simulink model "Adaptive_Control_KpKd"  (R2021b)
settings: Solver=VariableStepAuto  StartTime=0.0  StopTime=10  RelTol=1e-3
undefined symbols (not defined in the file or in its folder): coef_init, Kd, Kp, Kpi, Lambda, q_dq_init
(part 4 of 4)

== matlab function Adaptive_Control_KpKd/MATLAB Function1 ==
  data: q input; dq input; ddq input; Yb output; g input
function Yb = Yb_fun(q,dq,ddq,g)
%YB_FUN
%    YB = YB_FUN(Q1,Q2,Q3,Q4,Q5,Q6,DQ1,DQ2,DQ3,DQ4,DQ5,DQ6,DDQ1,DDQ2,DDQ3,DDQ4,DDQ5,DDQ6,G)

%    This function was generated by the Symbolic Math Toolbox version 8.7.
%    16-Mar-2022 17:09:26

q1 = q(1);
q2 = q(2);
q3 = q(3);
q4 = q(4);
q5 = q(5);
q6 = q(6);

dq1 = dq(1);
dq2 = dq(2);
dq3 = dq(3);
dq4 = dq(4);
dq5 = dq(5);
dq6 = dq(6);

ddq1 = ddq(1);
ddq2 = ddq(2);
ddq3 = ddq(3);
ddq4 = ddq(4);
ddq5 = ddq(5);
ddq6 = ddq(6);

t2 = cos(q1);
t3 = cos(q2);
t4 = cos(q4);
t5 = cos(q5);
t6 = cos(q6);
t7 = sin(q1);
t8 = sin(q2);
t9 = sin(q4);
t10 = sin(q5);
t11 = sin(q6);
t12 = dq1.^2;
t13 = dq2.^2;
t14 = dq4.^2;
t15 = dq5.^2;
t16 = dq6.^2;
t17 = q2.*2.0;
t18 = q4.*2.0;
t19 = q5.*2.0;
t20 = q6.*2.0;
t90 = q3.*5.0e+3;
t21 = cos(t17);
t22 = t3.^2;
t23 = t4.^2;
t24 = t5.^2;
t25 = t6.^2;
t26 = sin(t17);
t27 = sin(t18);
t28 = sin(t19);
t29 = sin(t20);
t30 = t8.^2;
t31 = t9.^2;
t32 = ddq1.*t3;
t33 = ddq2.*t3;
t34 = ddq2.*t4;
t35 = ddq4.*t5;
t36 = ddq5.*t4;
t37 = ddq5.*t5;
t38 = g.*t2;
t39 = ddq1.*t8;
t40 = ddq2.*t9;
t41 = ddq4.*t8;
t42 = ddq4.*t9;
t43 = ddq4.*t10;
t44 = ddq5.*t10;
t45 = dq2.*dq4.*t9;
t46 = dq2.*dq5.*t9;
t47 = dq4.*dq5.*t9;
t48 = dq1.*dq2.*t3;
t49 = dq1.*dq4.*t3;
t50 = dq2.*dq4.*t3;
t51 = dq4.*dq5.*t5;
t52 = dq4.*dq6.*t5;
t53 = dq5.*dq6.*t5;
t54 = t8.*t13;
t55 = t10.*t13;
t56 = t10.*t15;
t57 = dq2.*dq4.*t10.*2.0;
t58 = -t12;
t60 = ddq4.*t3.*t4;
t63 = ddq6.*t5.*t6;
t71 = ddq5.*t3.*t9;
t75 = ddq6.*t5.*t11;
t84 = g.*t7.*t8;
t98 = t4.*t12;
t99 = t5.*t13;
t100 = t4.*t14;
t101 = t5.*t15;
t102 = dq1.*dq2.*t4.*2.0;
t114 = dq1.*dq5.*t3.*t4;
t115 = dq2.*dq4.*t4.*t5;
t116 = dq4.*dq5.*t3.*t4;
t117 = dq2.*dq6.*t4.*t5;
t120 = dq1.*dq5.*t5.*t8;
t121 = dq1.*dq6.*t3.*t10;
t122 = dq1.*dq6.*t5.*t8;
t123 = dq2.*dq6.*t3.*t10;
t125 = dq1.*dq2.*t8.*t9;
t126 = dq1.*dq5.*t8.*t9;
t129 = dq2.*dq6.*t9.*t10;
t130 = dq5.*dq6.*t9.*t10;
t168 = t5.*t6.*t16;
t170 = dq1.*dq5.*t3.*t5.*2.0;
t171 = dq2.*dq5.*t4.*t5.*2.0;
t174 = t3.*t9.*t13;
t175 = t5.*t9.*t12;
t176 = t4.*t9.*t13;
t177 = t3.*t9.*t14;
t179 = t5.*t9.*t14;
t182 = t5.*t11.*t16;
t185 = dq1.*dq4.*t4.*t8.*2.0;
t186 = dq1.*dq2.*t5.*t9.*2.0;
t189 = dq2.*dq5.*t4.*t10.*2.0;
t196 = dq2.*dq3.*t9.*5.0e+3;
t207 = dq1.*dq2.*t4.*t5.*t8;
t211 = dq1.*dq6.*t3.*t5.*t9;
t215 = dq5.*dq6.*t3.*t4.*t10;
t277 = g.*t4.*t7.*2.5e+3;
t294 = dq2.*dq5.*t4.*t6.*t11.*2.0;
t295 = dq2.*dq6.*t4.*t6.*t11.*2.0;
t296 = dq5.*dq6.*t4.*t6.*t11.*2.0;
t297 = t3.*t8.*t9.*t12;
t305 = dq1.*dq4.*t5.*t8.*t9.*2.0;
t306 = dq1.*dq4.*t5.*t8.*t10.*2.0;
t307 = dq1.*dq5.*t3.*t9.*t10.*2.0;
t318 = dq1.*dq2.*t4.*t8.*7.8e+1;
t336 = dq2.*dq5.*t4.*t5.*t6.*-2.0;
t347 = dq1.*dq3.*t3.*t4.*5.0e+3;
t422 = t90-2.159e+3;
t425 = dq1.*dq2.*t4.*t8.*t90;
t455 = dq1.*dq5.*t3.*t6.*t9.*t11.*2.0;
t456 = dq1.*dq6.*t3.*t6.*t9.*t11.*2.0;
t459 = dq5.*dq6.*t3.*t6.*t9.*t11.*2.0;
t485 = dq1.*dq2.*q3.*t4.*t8.*-5.0e+3;
t490 = dq1.*dq4.*t4.*t5.*t8.*t10.*-2.0;
t519 = dq1.*dq6.*t3.*t4.*t6.*t9.*t11.*4.0;
t521 = dq2.*dq6.*t3.*t4.*t6.*t9.*t11.*4.0;
t59 = t4.*t32;
t61 = t5.*t34;
t62 = t4.*t35;
t64 = t3.*t38;
t65 = t9.*t32;
t66 = t10.*t32;
t67 = t5.*t39;
t68 = t10.*t33;
t69 = t10.*t34;
t70 = t5.*t40;
t72 = t6.*t40;
t73 = t8.*t37;
t74 = t6.*t44;
t76 = t8.*t38;
t77 = t9.*t39;
t78 = t10.*t39;
t79 = t8.*t40;
t80 = t10.*t40;
t81 = t11.*t40;
t82 = t9.*t44;
t83 = t11.*t44;
t85 = -t37;
t86 = -t38;
t87 = -t43;
t88 = -t44;
t89 = t40.*3.9e+1;
t91 = ddq1.*t22;
t92 = ddq1.*t24;
t93 = ddq2.*t23;
t94 = ddq2.*t24;
t95 = ddq2.*t25;
t96 = ddq4.*t24;
t97 = ddq5.*t25;
t103 = -t45;
t104 = -t47;
t105 = dq1.*dq2.*t26;
t106 = dq2.*dq4.*t27;
t107 = dq1.*dq5.*t28;
t108 = dq2.*dq5.*t28;
t109 = dq2.*dq6.*t29;
t110 = dq4.*dq5.*t28;
t111 = dq5.*dq6.*t29;
t113 = t4.*t49;
t118 = t4.*t52;
t119 = t10.*t48;
t124 = t8.*t53;
t127 = t8.*t46;
t128 = t10.*t46;
t131 = -t48;
t132 = -t49;
t133 = -t50;
t134 = -t51;
t135 = -t53;
t142 = t4.*t9.*t33;
t145 = t3.*t9.*t35;
t146 = t3.*t10.*t36;
t148 = t6.*t11.*t35;
t149 = t6.*t11.*t37;
t150 = t12.*t22;
t154 = t9.*t10.*t35;
t159 = -t71;
t163 = -t84;
t164 = t25.*t34;
t165 = t25.*t36;
t166 = t6.*t99;
t167 = t6.*t101;
t169 = t5.*t48.*2.0;
t172 = t24.*t39;
t173 = t24.*t41;
t178 = t11.*t99;
t180 = t9.*t101;
t181 = t11.*t101;
t183 = t8.*t48.*2.0;
t184 = t8.*t102;
t187 = t4.*t45.*2.0;
t188 = t4.*t57;
t190 = t10.*t54;
t191 = t8.*t56;
t195 = -t101;
t197 = q3.*t40.*2.5e+3;
t198 = t23.*t49;
t199 = t31.*t49;
t201 = t13.*t23.*2.0;
t208 = t5.*t9.*t49;
t209 = t10.*t114;
t210 = t4.*t121;
t212 = t4.*t122;
t213 = t8.*t117;
t214 = t3.*t9.*t52;
t217 = -t116;
t218 = -t171;
t219 = -t117;
t221 = -t120;
t222 = -t123;
t224 = -t125;
t225 = -t126;
t227 = -t130;
t240 = t23.*t48.*2.0;
t241 = t25.*t48.*2.0;
t242 = dq1.*dq2.*t4.*t22.*4.0;
t244 = t23.*t50.*2.0;
t245 = t25.*t49.*2.0;
t246 = t24.*t50.*2.0;
t247 = t25.*t50.*2.0;
t248 = t25.*t51.*2.0;
t249 = t25.*t52.*2.0;
t250 = t25.*t53.*2.0;
t257 = dq1.*dq4.*t10.*t22.*2.0;
t258 = t24.*t45.*2.0;
t259 = t25.*t45.*2.0;
t260 = t24.*t46.*2.0;
t261 = dq2.*dq4.*t10.*t23.*4.0;
t262 = t25.*t46.*2.0;
t263 = t24.*t47.*2.0;
t273 = t22.*t58;
t278 = t3.*t4.*t99;
t279 = t3.*t5.*t100;
t280 = t3.*t4.*t101;
t281 = t6.*t171;
t283 = t25.*t71;
t284 = t3.*t8.*t98;
t285 = t5.*t10.*t98;
t286 = t4.*t9.*t99;
t287 = t5.*t10.*t100;
t288 = t8.*t114.*2.0;
t289 = t4.*t9.*t48.*4.0;
t290 = t5.*t10.*t102;
t291 = t9.*t170;
t292 = t4.*t5.*t46.*2.0;
t293 = t11.*t171;
t298 = t4.*t9.*t54;
t299 = t4.*t9.*t55;
t300 = t6.*t11.*t55;
t301 = t6.*t11.*t56;
t302 = t8.*t9.*t49.*2.0;
t303 = t5.*t125.*2.0;
t304 = t9.*t10.*t49.*2.0;
t308 = t10.*t120.*2.0;
t309 = t8.*t189;
t310 = t4.*t129.*2.0;
t311 = t8.*t10.*t51.*2.0;
t312 = t6.*t11.*t57;
t317 = -t182;
t320 = t22.*t98.*2.0;
t326 = t23.*t55.*2.0;
t329 = (t12.*t26)./2.0;
t330 = (t12.*t28)./2.0;
t331 = (t13.*t27)./2.0;
t332 = (t13.*t28)./2.0;
t333 = (t13.*t29)./2.0;
t334 = (t14.*t28)./2.0;
t335 = (t15.*t29)./2.0;
t339 = -t207;
t344 = -t215;
t345 = -t306;
t346 = -t307;
t353 = t24.*t114.*2.0;
t354 = t23.*t170;
t355 = t25.*t114.*2.0;
t356 = dq2.*dq5.*t3.*t5.*t23.*2.0;
t357 = t24.*t116.*2.0;
t358 = t25.*t115.*2.0;
t359 = t25.*t117.*2.0;
t369 = t3.*t8.*t12.*t23;
t370 = t3.*t8.*t12.*t24;
t371 = t3.*t8.*t12.*t25;
t372 = t9.*t22.*t98;
t376 = t24.*t176;
t377 = t5.*t23.*t55;
t378 = t5.*t10.*t12.*t25;
t379 = t6.*t11.*t12.*t24;
t380 = t5.*t25.*t55;
t381 = t6.*t11.*t13.*t24;
t382 = t5.*t10.*t14.*t25;
t383 = t6.*t11.*t14.*t24;
t388 = dq1.*dq4.*t4.*t9.*t22.*2.0;
t390 = dq1.*dq2.*t5.*t9.*t22.*4.0;
t391 = dq1.*dq5.*t5.*t10.*t22.*2.0;
t392 = t23.*t121.*2.0;
t393 = t25.*t120.*2.0;
t395 = t23.*t123.*2.0;
t396 = t25.*t121.*2.0;
t397 = t25.*t122.*2.0;
t398 = dq1.*dq6.*t6.*t11.*t22.*2.0;
t399 = dq2.*dq5.*t5.*t10.*t23.*2.0;
t400 = t25.*t123.*2.0;
t401 = dq1.*dq5.*t5.*t10.*t25.*2.0;
t402 = t4.*t25.*t45.*4.0;
t403 = dq2.*dq5.*t5.*t10.*t25.*2.0;
t404 = dq1.*dq6.*t6.*t11.*t24.*2.0;
t406 = dq2.*dq6.*t6.*t11.*t24.*2.0;
t408 = dq2.*dq6.*t6.*t11.*t23.*4.0;
t409 = dq4.*dq6.*t6.*t11.*t24.*2.0;
t410 = t24.*t125.*2.0;
t411 = t24.*t126.*2.0;
t415 = t25.*t129.*2.0;
t416 = t25.*t130.*2.0;
t436 = t6.*t11.*t170;
t440 = t3.*t8.*t175;
t441 = t6.*t297;
t442 = t3.*t5.*t9.*t55;
t443 = t5.*t10.*t177;
t444 = t6.*t11.*t175;
t445 = t6.*t11.*t179;
t449 = t3.*t9.*t122.*2.0;
t450 = t5.*t10.*t185;
t453 = t3.*t4.*t10.*t45.*4.0;
t454 = t6.*t11.*t186;
t458 = t6.*t11.*t189;
t460 = t10.*t297;
t461 = t11.*t297;
t464 = t3.*t10.*t126.*2.0;
t465 = t3.*t4.*t8.*t58;
t466 = t4.*t5.*t10.*t58;
t468 = t3.*t8.*t9.*t58;
t470 = t297.*3.9e+1;
t475 = t25.*t176.*2.0;
t477 = t8.*t23.*t48.*-2.0;
t478 = t8.*t24.*t48.*-2.0;
t494 = t3.*t8.*t23.*t58;
t508 = t23.*t25.*t48.*4.0;
t512 = t23.*t25.*t50.*4.0;
t522 = dq1.*dq4.*t10.*t22.*t23.*4.0;
t534 = t6.*t11.*t305;
t535 = t6.*t11.*t307;
t537 = t5.*t6.*t10.*t11.*t45.*2.0;
t538 = t5.*t6.*t11.*t129.*2.0;
t539 = t6.*t9.*t10.*t11.*t52.*2.0;
t550 = t8.*t24.*t114.*4.0;
t551 = dq1.*dq5.*t4.*t5.*t9.*t22.*2.0;
t556 = t25.*t211.*2.0;
t560 = t25.*t215.*2.0;
t564 = dq1.*dq6.*t4.*t9.*t10.*t22.*2.0;
t565 = t25.*t306;
t567 = dq1.*dq4.*t6.*t8.*t11.*t24.*2.0;
t572 = t4.*t25.*t129.*4.0;
t574 = q3.*t297.*2.5e+3;
t576 = t23.*t24.*t48.*-2.0;
t585 = dq1.*dq2.*t4.*t5.*t10.*t22.*-4.0;
t614 = dq1.*dq4.*t4.*t9.*t22.*t25.*4.0;
t617 = t23.*t25.*t121.*4.0;
t619 = dq1.*dq6.*t6.*t11.*t22.*t23.*4.0;
t621 = t23.*t25.*t123.*4.0;
t632 = t6.*t9.*t10.*t11.*t122.*2.0;
t645 = t3.*t9.*t25.*t122.*4.0;
t653 = dq1.*dq4.*t4.*t9.*t22.*t24.*-2.0;
t654 = dq1.*dq5.*t5.*t10.*t22.*t23.*-2.0;
t664 = dq1.*dq6.*t4.*t9.*t10.*t22.*t25.*4.0;
t672 = t4.*t6.*t9.*t11.*t24.*t48.*2.0;
t677 = t3.*t9.*t24.*t295;
t112 = -t89;
t136 = t5.*t59;
t137 = t6.*t59;
t138 = t9.*t59;
t139 = t10.*t59;
t140 = t5.*t65;
t141 = t4.*t67;
t143 = t11.*t59;
t144 = t8.*t61;
t147 = t6.*t69;
t151 = t10.*t65;
t152 = t10.*t70;
t153 = t11.*t69;
t155 = -t61;
t156 = t59.*3.9e+1;
t157 = -t65;
t158 = -t69;
t160 = -t74;
t161 = -t78;
t162 = -t81;
t192 = -t91;
t193 = -t92;
t194 = -t96;
t200 = t8.*t59.*2.0;
t202 = t9.*t69.*2.0;
t203 = -t105;
t204 = -t106;
t205 = -t108;
t216 = -t113;
t220 = -t119;
t223 = -t124;
t226 = -t128;
t229 = t3.*t10.*t62;
t230 = t6.*t11.*t61;
t231 = t6.*t11.*t62;
t232 = t23.*t91;
t233 = t24.*t91;
t234 = t25.*t91;
t235 = t24.*t93;
t236 = t25.*t92;
t237 = t25.*t94;
t238 = t25.*t96;
t239 = t5.*t150;
t243 = t198.*2.0;
t252 = t6.*t11.*t66;
t253 = t6.*t11.*t67;
t254 = t6.*t11.*t68;
t255 = t6.*t11.*t73;
t256 = t10.*t150;
t264 = t9.*t10.*t67;
t267 = t10.*t11.*t72;
t268 = t9.*t11.*t74;
t270 = -t142;
t274 = -t201;
t276 = -t154;
t282 = t25.*t65;
t313 = -t167;
t314 = -t172;
t315 = -t173;
t316 = -t178;
t319 = t25.*t93.*2.0;
t321 = -t240;
t323 = -t244;
t324 = -t246;
t327 = -t260;
t328 = -t263;
t337 = t23.*t66.*2.0;
t338 = t23.*t68.*2.0;
t340 = t5.*t9.*t132;
t341 = -t209;
t342 = -t213;
t343 = -t214;
t348 = q3.*t59.*2.5e+3;
t350 = t23.*t169;
t351 = t24.*t113.*2.0;
t352 = t25.*t113.*2.0;
t360 = t25.*t118.*2.0;
t365 = t6.*t11.*t145;
t366 = t6.*t11.*t146;
t367 = t25.*t172;
t368 = t25.*t173;
t375 = t6.*t11.*t150;
t384 = t23.*t183;
t385 = t24.*t183;
t386 = t25.*t183;
t387 = t23.*t119.*2.0;
t389 = t25.*t119.*2.0;
t394 = t24.*t187;
t405 = t25.*t124.*2.0;
t407 = t10.*t248;
t412 = t24.*t127.*2.0;
t413 = t25.*t127.*2.0;
t414 = t25.*t128.*2.0;
t421 = t5.*t273;
t426 = t9.*t76.*2.5e+3;
t427 = -t329;
t428 = -t330;
t429 = -t334;
t431 = t24.*t142;
t432 = t5.*t284;
t433 = t5.*t8.*t113.*2.0;
t434 = t6.*t11.*t169;
t435 = t6.*t291;
t438 = t25.*t154;
t439 = t10.*t284;
t446 = t9.*t11.*t167;
t447 = t5.*t10.*t184;
t448 = t4.*t9.*t119.*4.0;
t451 = t9.*t10.*t113.*4.0;
t452 = t11.*t291;
t457 = t6.*t11.*t188;
t462 = t6.*t11.*t190;
t463 = t6.*t11.*t191;
t467 = -t287;
t469 = -t298;
t471 = -t353;
t472 = -t357;
t476 = t6.*t11.*t201;
t479 = -t388;
t480 = -t391;
t482 = t23.*t190.*2.0;
t483 = -t411;
t487 = t25.*t142.*2.0;
t488 = t23.*t150.*2.0;
t489 = t4.*t9.*t10.*t91.*2.0;
t491 = -t470;
t495 = t4.*t9.*t273;
t496 = -t376;
t497 = -t377;
t500 = t3.*t4.*t11.*t166;
t501 = t6.*t11.*t279;
t502 = t3.*t4.*t11.*t167;
t506 = t24.*t240;
t509 = t24.*t244;
Yb = ft_1({ddq1,ddq2,ddq3,ddq4,ddq5,ddq6,dq1,dq2,dq3,dq4,dq5,dq6,g,q3,t10,t100,t101,t102,t103,t104,t105,t106,t107,t108,t109,t11,t110,t111,t112,t113,t114,t115,t116,t117,t118,t119,t12,t120,t121,t122,t123,t124,t125,t126,t127,t128,t129,t13,t130,t131,t132,t133,t134,t135,t136,t137,t138,t139,t14,t140,t141,t142,t143,t144,t145,t146,t147,t148,t149,t15,t150,t151,t152,t153,t154,t155,t156,t157,t158,t159,t16,t160,t161,t162,t163,t164,t165,t166,t167,t168,t169,t170,t172,t173,t174,t175,t176,t177,t178,t179,t180,t181,t182,t183,t184,t185,t186,t187,t188,t189,t190,t191,t192,t193,t194,t195,t196,t197,t198,t199,t200,t201,t202,t203,t204,t205,t207,t208,t209,t21,t210,t211,t212,t213,t214,t215,t216,t217,t218,t219,t22,t220,t221,t222,t223,t224,t225,t226,t227,t229,t23,t230,t231,t232,t233,t234,t235,t236,t237,t238,t239,t24,t240,t241,t242,t243,t244,t245,t246,t247,t248,t249,t25,t250,t252,t253,t254,t255,t256,t257,t258,t259,t26,t260,t261,t262,t263,t264,t267,t268,t270,t273,t274,t276,t277,t278,t279,t28,t280,t282,t283,t284,t285,t286,t287,t288,t289,t29,t290,t291,t292,t293,t294,t295,t296,t297,t298,t299,t3,t30,t300,t301,t302,t303,t304,t305,t306,t307,t308,t309,t31,t310,t311,t312,t313,t314,t315,t316,t317,t318,t319,t32,t320,t321,t323,t324,t326,t327,t328,t329,t33,t330,t331,t332,t333,t334,t335,t336,t337,t338,t339,t34,t340,t341,t342,t343,t344,t345,t346,t347,t348,t35,t350,t351,t352,t353,t354,t355,t356,t357,t358,t359,t36,t360,t365,t366,t367,t368,t369,t37,t370,t371,t372,t375,t376,t377,t378,t379,t38,t380,t381,t382,t383,t384,t385,t386,t387,t388,t389,t39,t390,t391,t392,t393,t394,t395,t396,t397,t398,t399,t4,t40,t400,t401,t402,t403,t404,t405,t406,t407,t408,t409,t41,t410,t411,t412,t413,t414,t415,t416,t42,t421,t422,t426,t427,t428,t429,t43,t431,t432,t433,t434,t435,t436,t438,t439,t440,t441,t442,t443,t444,t445,t446,t447,t448,t449,t45,t450,t451,t452,t453,t454,t455,t456,t457,t458,t459,t46,t460,t461,t462,t463,t464,t465,t466,t467,t468,t469,t47,t471,t472,t475,t476,t477,t478,t479,t48,t480,t482,t483,t485,t487,t488,t489,t49,t490,t491,t494,t495,t496,t497,t5,t50,t500,t501,t502,t506,t508,t509,t51,t512,t519,t52,t521,t522,t53,t534,t535,t537,t538,t539,t54,t55,t550,t551,t556,t56,t560,t564,t565,t567,t57,t572,t574,t576,t58,t585,t59,t6,t60,t61,t614,t617,t619,t62,t621,t63,t632,t64,t645,t65,t653,t654,t66,t664,t67,t672,t677,t68,t69,t7,t70,t71,t72,t73,t74,t75,t76,t77,t78,t79,t8,t80,t81,t82,t83,t84,t85,t86,t87,t88,t9,t90,t91,t92,t93,t94,t95,t96,t97,t98,t99});
end
function Yb = ft_1(ct)
ddq1 = ct{1};
ddq2 = ct{2};
ddq3 = ct{3};
ddq4 = ct{4};
ddq5 = ct{5};
ddq6 = ct{6};
dq1 = ct{7};
dq2 = ct{8};
dq3 = ct{9};
dq4 = ct{10};
dq5 = ct{11};
dq6 = ct{12};
g = ct{13};
q3 = ct{14};
t10 = ct{15};
t100 = ct{16};
t101 = ct{17};
t102 = ct{18};
t103 = ct{19};
t104 = ct{20};
t105 = ct{21};
t106 = ct{22};
t107 = ct{23};
t108 = ct{24};
t109 = ct{25};
t11 = ct{26};
t110 = ct{27};
t111 = ct{28};
t112 = ct{29};
t113 = ct{30};
t114 = ct{31};
t115 = ct{32};
t116 = ct{33};
t117 = ct{34};
t118 = ct{35};
t119 = ct{36};
t12 = ct{37};
t120 = ct{38};
t121 = ct{39};
t122 = ct{40};
t123 = ct{41};
t124 = ct{42};
t125 = ct{43};
t126 = ct{44};
t127 = ct{45};
t128 = ct{46};
t129 = ct{47};
t13 = ct{48};
t130 = ct{49};
t131 = ct{50};
t132 = ct{51};
t133 = ct{52};
t134 = ct{53};
t135 = ct{54};
t136 = ct{55};
t137 = ct{56};
t138 = ct{57};
t139 = ct{58};
t14 = ct{59};
t140 = ct{60};
t141 = ct{61};
t142 = ct{62};
t143 = ct{63};
t144 = ct{64};
t145 = ct{65};
t146 = ct{66};
t147 = ct{67};
t148 = ct{68};
t149 = ct{69};
t15 = ct{70};
t150 = ct{71};
t151 = ct{72};
t152 = ct{73};
t153 = ct{74};
t154 = ct{75};
t155 = ct{76};
t156 = ct{77};
t157 = ct{78};
t158 = ct{79};
t159 = ct{80};
t16 = ct{81};
t160 = ct{82};
t161 = ct{83};
t162 = ct{84};
t163 = ct{85};
t164 = ct{86};
t165 = ct{87};
t166 = ct{88};
t167 = ct{89};
t168 = ct{90};
t169 = ct{91};
t170 = ct{92};
t172 = ct{93};
t173 = ct{94};
t174 = ct{95};
t175 = ct{96};
t176 = ct{97};
t177 = ct{98};
t178 = ct{99};
t179 = ct{100};
t180 = ct{101};
t181 = ct{102};
t182 = ct{103};
t183 = ct{104};
t184 = ct{105};
t185 = ct{106};
t186 = ct{107};
t187 = ct{108};
t188 = ct{109};
t189 = ct{110};
t190 = ct{111};
t191 = ct{112};
t192 = ct{113};
t193 = ct{114};
t194 = ct{115};
t195 = ct{116};
t196 = ct{117};
t197 = ct{118};
t198 = ct{119};
t199 = ct{120};
t200 = ct{121};
t201 = ct{122};
t202 = ct{123};
t203 = ct{124};
t204 = ct{125};
t205 = ct{126};
t207 = ct{127};
t208 = ct{128};
t209 = ct{129};
t21 = ct{130};
t210 = ct{131};
t211 = ct{132};
t212 = ct{133};
t213 = ct{134};
t214 = ct{135};
t215 = ct{136};
t216 = ct{137};
t217 = ct{138};
t218 = ct{139};
t219 = ct{140};
t22 = ct{141};
t220 = ct{142};
t221 = ct{143};
t222 = ct{144};
t223 = ct{145};
t224 = ct{146};
t225 = ct{147};
t226 = ct{148};
t227 = ct{149};
t229 = ct{150};
t23 = ct{151};
t230 = ct{152};
t231 = ct{153};
t232 = ct{154};
t233 = ct{155};
t234 = ct{156};
t235 = ct{157};
t236 = ct{158};
t237 = ct{159};
t238 = ct{160};
t239 = ct{161};
t24 = ct{162};
t240 = ct{163};
t241 = ct{164};
t242 = ct{165};
t243 = ct{166};
t244 = ct{167};
t245 = ct{168};
t246 = ct{169};
t247 = ct{170};
t248 = ct{171};
t249 = ct{172};
t25 = ct{173};
t250 = ct{174};
t252 = ct{175};
t253 = ct{176};
t254 = ct{177};
t255 = ct{178};
t256 = ct{179};
t257 = ct{180};
t258 = ct{181};
t259 = ct{182};
t26 = ct{183};
t260 = ct{184};
t261 = ct{185};
t262 = ct{186};
t263 = ct{187};
t264 = ct{188};
t267 = ct{189};
t268 = ct{190};
t270 = ct{191};
t273 = ct{192};
t274 = ct{193};
t276 = ct{194};
t277 = ct{195};
t278 = ct{196};
t279 = ct{197};
t28 = ct{198};
t280 = ct{199};
t282 = ct{200};
t283 = ct{201};
t284 = ct{202};
t285 = ct{203};
t286 = ct{204};
t287 = ct{205};
t288 = ct{206};
t289 = ct{207};
t29 = ct{208};
t290 = ct{209};
t291 = ct{210};
t292 = ct{211};
t293 = ct{212};
t294 = ct{213};
t295 = ct{214};
t296 = ct{215};
t297 = ct{216};
t298 = ct{217};
t299 = ct{218};
t3 = ct{219};
t30 = ct{220};
t300 = ct{221};
t301 = ct{222};
t302 = ct{223};
t303 = ct{224};
t304 = ct{225};
t305 = ct{226};
t306 = ct{227};
t307 = ct{228};
t308 = ct{229};
t309 = ct{230};
t31 = ct{231};
t310 = ct{232};
t311 = ct{233};
t312 = ct{234};
t313 = ct{235};
t314 = ct{236};
t315 = ct{237};
t316 = ct{238};
t317 = ct{239};
t318 = ct{240};
t319 = ct{241};
t32 = ct{242};
t320 = ct{243};
t321 = ct{244};
t323 = ct{245};
t324 = ct{246};
t326 = ct{247};
t327 = ct{248};
t328 = ct{249};
t329 = ct{250};
t33 = ct{251};
t330 = ct{252};
t331 = ct{253};
t332 = ct{254};
t333 = ct{255};
t334 = ct{256};
t335 = ct{257};
t336 = ct{258};
t337 = ct{259};
t338 = ct{260};
t339 = ct{261};
t34 = ct{262};
t340 = ct{263};
t341 = ct{264};
t342 = ct{265};
t343 = ct{266};
t344 = ct{267};
t345 = ct{268};
t346 = ct{269};
t347 = ct{270};
t348 = ct{271};
t35 = ct{272};
t350 = ct{273};
t351 = ct{274};
t352 = ct{275};
t353 = ct{276};
t354 = ct{277};
t355 = ct{278};
t356 = ct{279};
t357 = ct{280};
t358 = ct{281};
t359 = ct{282};
t36 = ct{283};
t360 = ct{284};
t365 = ct{285};
t366 = ct{286};
t367 = ct{287};
t368 = ct{288};
t369 = ct{289};
t37 = ct{290};
t370 = ct{291};
t371 = ct{292};
t372 = ct{293};
t375 = ct{294};
t376 = ct{295};
t377 = ct{296};
t378 = ct{297};
t379 = ct{298};
t38 = ct{299};
t380 = ct{300};
t381 = ct{301};
t382 = ct{302};
t383 = ct{303};
t384 = ct{304};
t385 = ct{305};
t386 = ct{306};
t387 = ct{307};
t388 = ct{308};
t389 = ct{309};
t39 = ct{310};
t390 = ct{311};
t391 = ct{312};
t392 = ct{313};
t393 = ct{314};
t394 = ct{315};
t395 = ct{316};
t396 = ct{317};
t397 = ct{318};
t398 = ct{319};
t399 = ct{320};
t4 = ct{321};
t40 = ct{322};
t400 = ct{323};
t401 = ct{324};
t402 = ct{325};
t403 = ct{326};
t404 = ct{327};
t405 = ct{328};
t406 = ct{329};
t407 = ct{330};
t408 = ct{331};
t409 = ct{332};
t41 = ct{333};
t410 = ct{334};
t411 = ct{335};
t412 = ct{336};
t413 = ct{337};
t414 = ct{338};
t415 = ct{339};
t416 = ct{340};
t42 = ct{341};
t421 = ct{342};
t422 = ct{343};
t426 = ct{344};
t427 = ct{345};
t428 = ct{346};
t429 = ct{347};
t43 = ct{348};
t431 = ct{349};
t432 = ct{350};
t433 = ct{351};
t434 = ct{352};
t435 = ct{353};
t436 = ct{354};
t438 = ct{355};
t439 = ct{356};
t440 = ct{357};
t441 = ct{358};
t442 = ct{359};
t443 = ct{360};
t444 = ct{361};
t445 = ct{362};
t446 = ct{363};
t447 = ct{364};
t448 = ct{365};
t449 = ct{366};
t45 = ct{367};
t450 = ct{368};
t451 = ct{369};
t452 = ct{370};
t453 = ct{371};
t454 = ct{372};
t455 = ct{373};
t456 = ct{374};
t457 = ct{375};
t458 = ct{376};
t459 = ct{377};
t46 = ct{378};
t460 = ct{379};
t461 = ct{380};
t462 = ct{381};
t463 = ct{382};
t464 = ct{383};
t465 = ct{384};
t466 = ct{385};
t467 = ct{386};
t468 = ct{387};
t469 = ct{388};
t47 = ct{389};
t471 = ct{390};
t472 = ct{391};
t475 = ct{392};
t476 = ct{393};
t477 = ct{394};
t478 = ct{395};
t479 = ct{396};
t48 = ct{397};
t480 = ct{398};
t482 = ct{399};
t483 = ct{400};
t485 = ct{401};
t487 = ct{402};
t488 = ct{403};
t489 = ct{404};
t49 = ct{405};
t490 = ct{406};
t491 = ct{407};
t494 = ct{408};
t495 = ct{409};
t496 = ct{410};
t497 = ct{411};
t5 = ct{412};
t50 = ct{413};
t500 = ct{414};
t501 = ct{415};
t502 = ct{416};
t506 = ct{417};
t508 = ct{418};
t509 = ct{419};
t51 = ct{420};
t512 = ct{421};
t519 = ct{422};
t52 = ct{423};
t521 = ct{424};
t522 = ct{425};
t53 = ct{426};
t534 = ct{427};
t535 = ct{428};
t537 = ct{429};
t538 = ct{430};
t539 = ct{431};
t54 = ct{432};
t55 = ct{433};
t550 = ct{434};
t551 = ct{435};
t556 = ct{436};
t56 = ct{437};
t560 = ct{438};
t564 = ct{439};
t565 = ct{440};
t567 = ct{441};
t57 = ct{442};
t572 = ct{443};
t574 = ct{444};
t576 = ct{445};
t58 = ct{446};
t585 = ct{447};
t59 = ct{448};
t6 = ct{449};
t60 = ct{450};
t61 = ct{451};
t614 = ct{452};
t617 = ct{453};
t619 = ct{454};
t62 = ct{455};
t621 = ct{456};
t63 = ct{457};
t632 = ct{458};
t64 = ct{459};
t645 = ct{460};
t65 = ct{461};
t653 = ct{462};
t654 = ct{463};
t66 = ct{464};
t664 = ct{465};
t67 = ct{466};
t672 = ct{467};
t677 = ct{468};
t68 = ct{469};
t69 = ct{470};
t7 = ct{471};
t70 = ct{472};
t71 = ct{473};
t72 = ct{474};
t73 = ct{475};
t74 = ct{476};
t75 = ct{477};
t76 = ct{478};
t77 = ct{479};
t78 = ct{480};
t79 = ct{481};
t8 = ct{482};
t80 = ct{483};
t81 = ct{484};
t82 = ct{485};
t83 = ct{486};
t84 = ct{487};
t85 = ct{488};
t86 = ct{489};
t87 = ct{490};
t88 = ct{491};
t9 = ct{492};
t90 = ct{493};
t91 = ct{494};
t92 = ct{495};
t93 = ct{496};
t94 = ct{497};
t95 = ct{498};
t96 = ct{499};
t97 = ct{500};
t98 = ct{501};
t99 = ct{502};
t510 = t25.*t198.*4.0;
t511 = t25.*t246;
t514 = t4.*t9.*t11.*t166;
t515 = t4.*t5.*t9.*t119.*2.0;
t516 = t5.*t9.*t209.*2.0;
t517 = t6.*t11.*t289;
t518 = t3.*t4.*t5.*t128.*2.0;
t520 = t6.*t11.*t292;
t523 = t25.*t258;
t524 = t25.*t260;
t525 = t25.*t263;
t528 = t10.*t440;
t531 = t8.*t10.*t208.*2.0;
t532 = t6.*t11.*t303;
t533 = t6.*t11.*t304;
t536 = t6.*t11.*t309;
t540 = t5.*t468;
t541 = t6.*t468;
t542 = -t442;
t543 = t25.*t284;
t544 = t5.*t372;
t545 = t25.*t285;
t546 = t25.*t287;
t547 = t5.*t25.*t184;
t548 = t25.*t288;
t549 = t5.*t10.*t242;
t552 = t25.*t208.*2.0;
t553 = t25.*t290;
t554 = t25.*t209.*2.0;
t555 = t25.*t210.*2.0;
t557 = t25.*t212.*2.0;
t558 = t25.*t213.*2.0;
t559 = t25.*t214.*2.0;
t561 = t10.*t372;
t562 = t24.*t298;
t566 = t6.*t11.*t257;
t568 = t25.*t308;
t569 = t8.*t404;
t571 = t6.*t11.*t261;
t573 = t8.*t409;
t583 = t24.*t284.*2.0;
t584 = t22.*t285.*2.0;
t586 = -t550;
t588 = t25.*t298.*2.0;
t589 = t25.*t299.*2.0;
t590 = t23.*t300.*2.0;
t592 = t25.*t353;
t593 = t25.*t357;
t596 = t5.*t6.*t10.*t11.*t113.*2.0;
t597 = t5.*t6.*t11.*t210.*2.0;
t598 = t3.*t6.*t10.*t11.*t118.*2.0;
t599 = t24.*t369;
t600 = t25.*t370;
t601 = t24.*t372;
t605 = t25.*t376;
t606 = t25.*t377;
t607 = t23.*t381;
t610 = t8.*t508;
t611 = t24.*t388;
t612 = t23.*t25.*t119.*4.0;
t613 = t23.*t391;
t615 = t25.*t391;
t618 = t24.*t398;
t620 = t25.*t399;
t622 = t23.*t406;
t625 = t6.*t11.*t453;
t626 = t25.*t410;
t627 = t25.*t411;
t629 = t10.*t11.*t441;
t631 = t6.*t11.*t464;
t633 = t8.*t538;
t638 = t6.*t11.*t354;
t639 = t6.*t11.*t356;
t640 = t3.*t9.*t380;
t641 = t25.*t443;
t643 = t25.*t450;
t644 = t6.*t11.*t390;
t649 = t25.*t369.*2.0;
t650 = t9.*t25.*t320;
t652 = t24.*t477;
t656 = t25.*t440.*2.0;
t660 = t25.*t550;
t661 = t5.*t6.*t8.*t11.*t210.*4.0;
t663 = t6.*t11.*t522;
t674 = t6.*t11.*t551;
t676 = t3.*t4.*t9.*t404;
t206 = -t156;
t228 = t10.*t136;
t251 = t6.*t151;
t265 = t11.*t151;
t266 = t8.*t152;
t269 = -t138;
t271 = -t143;
t272 = -t147;
t275 = -t152;
t322 = -t243;
t325 = t8.*t140.*2.0;
t349 = t6.*t239;
t361 = t10.*t11.*t137;
t362 = t6.*t11.*t140;
t363 = t6.*t11.*t141;
t364 = t6.*t11.*t144;
t373 = t10.*t239;
t374 = t11.*t239;
t418 = -t229;
t419 = t23.*t192;
t420 = -t235;
t423 = -t264;
t430 = t24.*t138;
t437 = t25.*t152;
t474 = t9.*t239.*2.0;
t481 = t9.*t11.*t147.*2.0;
t484 = -t412;
t486 = t25.*t138.*2.0;
t492 = t6.*t421;
t499 = t25.*t229;
t503 = t24.*t232;
t504 = t25.*t233;
t505 = t25.*t235;
t507 = t24.*t243;
t513 = t6.*t439;
t526 = t25.*t264;
t529 = t11.*t439;
t530 = t8.*t448;
t563 = t6.*t11.*t256;
t570 = t8.*t407;
t575 = t25.*t232.*2.0;
t577 = t23.*t252.*2.0;
t578 = t23.*t254.*2.0;
t579 = -t516;
t580 = -t518;
t581 = t23.*t256.*2.0;
t582 = t9.*t439.*2.0;
t591 = t25.*t351;
t594 = t6.*t11.*t432;
t595 = t6.*t11.*t433;
t604 = t24.*t375;
t608 = t24.*t384;
t609 = t25.*t385;
t616 = t25.*t394;
t623 = t6.*t11.*t448;
t624 = t6.*t11.*t451;
t628 = t25.*t412;
t630 = t10.*t532;
t634 = t10.*t540;
t636 = t25.*t431;
t637 = t6.*t11.*t350;
t642 = t25.*t447;
t646 = t10.*t495;
t647 = t24.*t469;
t651 = t23.*t375.*2.0;
t655 = t6.*t11.*t489;
t658 = t23.*t462.*2.0;
t659 = t25.*t549;
t662 = t25.*t562;
t667 = t25.*t506;
t669 = t25.*t509;
t670 = t6.*t11.*t544;
t671 = t4.*t5.*t9.*t389;
t673 = t25.*t516;
t675 = t3.*t4.*t5.*t414;
t678 = t25.*t528;
t679 = t25.*t531;
t680 = t24.*t543.*2.0;
t681 = t22.*t545.*2.0;
t683 = t10.*t650;
t686 = t25.*t599;
t687 = t25.*t601;
t691 = t25.*t611;
t692 = t25.*t613;
t693 = t23.*t618;
t417 = -t228;
t424 = -t266;
t473 = t8.*t228.*2.0;
t498 = t25.*t228;
t527 = t25.*t266;
t587 = t6.*t11.*t325;
t602 = t23.*t373;
t603 = t25.*t373;
t635 = t25.*t430;
t657 = t9.*t11.*t349.*2.0;
t665 = t6.*t11.*t530;
t666 = t25.*t503;
t668 = t25.*t507;
t682 = t10.*t594.*2.0;
t684 = t23.*t563.*2.0;
t685 = t9.*t11.*t513.*2.0;
t689 = t23.*t604;
t690 = t25.*t608;
t694 = t112+t196+t197+t206+t277+t318+t347+t348+t426+t485+t491+t574;
t493 = -t473;
t648 = t25.*t473;
t688 = t25.*t602;
et1 = ddq1.*t6.*1.82e-2+t6.*t41.*1.82e-2+t6.*t50.*3.64e-2-t6.*t71.*1.82e-2-t11.*t68.*9.1e-3+t11.*t73.*9.1e-3-t6.*t92.*1.82e-2-t6.*t123.*1.82e-2+t6.*t127.*3.64e-2-t6.*t142.*1.82e-2+t11.*t144.*9.1e-3-t11.*t145.*9.1e-3+t11.*t146.*9.1e-3-t6.*t173.*1.82e-2+t11.*t190.*9.1e-3-t11.*t191.*9.1e-3;
et2 = t6.*t214.*(-1.82e-2)-t6.*t229.*1.82e-2-t6.*t232.*1.82e-2+t6.*t233.*1.82e-2-t6.*t266.*1.82e-2-t11.*t279.*9.1e-3+t6.*t298.*1.82e-2+t6.*t431.*1.82e-2-t6.*t442.*1.82e-2+t6.*t443.*1.82e-2+t6.*t503.*1.82e-2-t6.*t562.*1.82e-2-dq1.*dq6.*t11.*1.82e-2+t4.*t11.*t38-t8.*t11.*t34.*1.56e-2+t3.*t11.*t42.*1.56e-2+t3.*t4.*t63.*9.1e-3;
et3 = t6.*t23.*t50.*(-3.64e-2)-t6.*t24.*t50.*3.64e-2+t8.*t11.*t65.*3.12e-2+t8.*t10.*t72.*1.56e-2-t5.*t6.*t91.*3.12e-2+t11.*t23.*t68.*1.82e-2+t3.*t11.*t100.*1.56e-2+t6.*t8.*t114.*3.64e-2+t8.*t11.*t113.*3.12e-2-t6.*t24.*t116.*3.64e-2+t6.*t23.*t123.*1.82e-2+t8.*t10.*t137.*3.12e-2-t6.*t24.*t127.*3.64e-2-t8.*t11.*t140.*1.82e-2+t9.*t11.*t163+t3.*t4.*t178.*9.1e-3+t3.*t4.*t181.*9.1e-3;
et4 = t3.*t4.*t182.*(-9.1e-3)-t6.*t10.*t177.*1.56e-2-t11.*t23.*t190.*1.82e-2-t8.*t11.*t210.*3.12e-2-t6.*t8.*t228.*3.64e-2-dq1.*dq2.*t9.*t11.*3.12e-2-dq4.*dq6.*t8.*t11.*1.82e-2+dq1.*dq6.*t11.*t24.*1.82e-2-ddq6.*t3.*t4.*t6.*1.56e-2-ddq3.*t3.*t4.*t11-ddq6.*t6.*t8.*t10.*9.1e-3+q3.*t8.*t11.*t34-q3.*t3.*t11.*t42-q3.*t8.*t11.*t65.*2.0-q3.*t8.*t10.*t72+q3.*t5.*t6.*t91.*2.0-q3.*t3.*t11.*t100+q3.*t6.*t10.*t102-q3.*t8.*t11.*t113.*2.0-q3.*t8.*t10.*t137.*2.0;
et5 = q3.*t6.*t10.*t177+q3.*t8.*t11.*t210.*2.0+q3.*t6.*t10.*t302-t3.*t4.*t11.*t13.*1.56e-2+t3.*t4.*t11.*t16.*1.56e-2+t8.*t10.*t11.*t16.*9.1e-3+t3.*t6.*t9.*t37.*1.56e-2+t3.*t4.*t6.*t43.*1.56e-2+t3.*t4.*t6.*t51.*3.12e-2+t5.*t6.*t8.*t48.*(3.9e+1./6.25e+2)+t3.*t6.*t9.*t55.*1.56e-2-t3.*t6.*t9.*t56.*1.56e-2+t6.*t8.*t10.*t51.*3.64e-2-t3.*t9.*t11.*t53.*3.12e-2+t6.*t8.*t23.*t48.*3.64e-2-t6.*t8.*t24.*t48.*3.64e-2+t6.*t23.*t24.*t50.*3.64e-2+t6.*t9.*t10.*t86;
et6 = t5.*t6.*t8.*t114.*3.12e-2-t5.*t8.*t11.*t113.*1.82e-2-t3.*t6.*t9.*t122.*1.82e-2+t3.*t10.*t11.*t118.*1.82e-2+t3.*t10.*t11.*t126.*1.82e-2-t6.*t8.*t24.*t114.*7.28e-2+t5.*t8.*t11.*t129.*1.82e-2+t4.*t6.*t10.*t163+t6.*t8.*t10.*t208.*3.64e-2+t5.*t8.*t11.*t210.*3.64e-2+dq1.*dq2.*q3.*t9.*t11.*2.0-dq1.*dq2.*t4.*t6.*t10.*3.12e-2+dq1.*dq5.*t5.*t6.*t10.*3.64e-2+dq1.*dq2.*t5.*t9.*t11.*1.82e-2+dq2.*dq3.*t4.*t8.*t11.*2.0+dq4.*dq6.*t3.*t6.*t9.*3.12e-2;
et7 = dq5.*dq6.*t3.*t9.*t11.*1.82e-2+dq1.*dq3.*t5.*t6.*t22.*2.0+dq1.*dq5.*t6.*t10.*t22.*3.12e-2+dq1.*dq2.*t9.*t11.*t22.*(3.9e+1./6.25e+2)+dq1.*dq6.*t5.*t11.*t22.*3.12e-2+dq1.*dq4.*t10.*t11.*t22.*1.82e-2+dq4.*dq6.*t8.*t11.*t24.*1.82e-2+dq1.*dq6.*t11.*t22.*t23.*1.82e-2-dq1.*dq6.*t11.*t22.*t24.*1.82e-2+ddq6.*q3.*t3.*t4.*t6+ddq3.*t3.*t6.*t9.*t10-ddq6.*t3.*t9.*t10.*t11.*1.56e-2+g.*t3.*t5.*t6.*t7+q3.*t3.*t4.*t11.*t13-q3.*t3.*t4.*t11.*t16-q3.*t3.*t4.*t6.*t51.*2.0-q3.*t5.*t6.*t8.*t48.*4.0-q3.*t3.*t6.*t9.*t55+q3.*t3.*t6.*t9.*t56+q3.*t3.*t9.*t11.*t53.*2.0;
et8 = q3.*t3.*t4.*t6.*t87+q3.*t3.*t6.*t9.*t85-q3.*t5.*t6.*t8.*t114.*2.0-t3.*t6.*t9.*t10.*t16.*1.56e-2-t3.*t4.*t10.*t11.*t45.*3.64e-2-t6.*t8.*t9.*t10.*t49.*3.12e-2-t6.*t8.*t23.*t24.*t48.*3.64e-2-t4.*t9.*t10.*t11.*t91.*1.82e-2-t3.*t4.*t5.*t6.*t128.*3.64e-2+t4.*t8.*t9.*t11.*t119.*3.64e-2+ddq6.*q3.*t3.*t9.*t10.*t11+q3.*t3.*t6.*t9.*t10.*t16-dq4.*dq6.*q3.*t3.*t6.*t9.*2.0-dq1.*dq5.*q3.*t6.*t10.*t22.*2.0-dq1.*dq2.*q3.*t9.*t11.*t22.*4.0-dq1.*dq6.*q3.*t5.*t11.*t22.*2.0+dq1.*dq2.*t4.*t5.*t6.*t10.*3.64e-2;
et9 = dq1.*dq6.*t3.*t6.*t8.*t9.*3.12e-2-dq1.*dq3.*t3.*t8.*t9.*t11.*2.0+dq2.*dq6.*t3.*t4.*t9.*t11.*1.82e-2-dq2.*dq3.*t6.*t8.*t9.*t10.*2.0-dq4.*dq6.*t3.*t4.*t10.*t11.*3.12e-2-dq2.*dq5.*t4.*t8.*t10.*t11.*1.82e-2+dq1.*dq2.*t4.*t6.*t10.*t22.*(3.9e+1./6.25e+2)+dq1.*dq4.*t4.*t6.*t9.*t22.*3.64e-2-dq1.*dq5.*t5.*t6.*t10.*t22.*3.64e-2+dq2.*dq5.*t3.*t5.*t11.*t23.*1.82e-2-dq1.*dq2.*t5.*t9.*t11.*t22.*3.64e-2-dq1.*dq4.*t10.*t11.*t22.*t23.*3.64e-2-dq1.*dq6.*t11.*t22.*t23.*t24.*1.82e-2-dq1.*dq6.*q3.*t3.*t6.*t8.*t9.*2.0;
et10 = dq4.*dq6.*q3.*t3.*t4.*t10.*t11.*2.0-dq1.*dq2.*q3.*t4.*t6.*t10.*t22.*4.0-dq1.*dq3.*t3.*t4.*t6.*t8.*t10.*2.0-dq1.*dq2.*t4.*t5.*t6.*t10.*t22.*7.28e-2-dq1.*dq5.*t4.*t5.*t9.*t11.*t22.*1.82e-2-dq1.*dq6.*t4.*t6.*t9.*t10.*t22.*1.82e-2-dq2.*dq6.*t3.*t4.*t9.*t11.*t24.*1.82e-2-dq1.*dq4.*t4.*t6.*t9.*t22.*t24.*3.64e-2-dq1.*dq5.*t5.*t6.*t10.*t22.*t23.*3.64e-2;
et11 = ddq1.*t11.*1.82e-2+t11.*t41.*1.82e-2+t11.*t50.*3.64e-2+t6.*t68.*9.1e-3-t6.*t73.*9.1e-3-t11.*t71.*1.82e-2-t11.*t92.*1.82e-2-t11.*t123.*1.82e-2+t11.*t127.*3.64e-2-t6.*t144.*9.1e-3+t6.*t145.*9.1e-3-t6.*t146.*9.1e-3-t11.*t142.*1.82e-2-t11.*t173.*1.82e-2-t6.*t190.*9.1e-3+t6.*t191.*9.1e-3;
et12 = t11.*t214.*(-1.82e-2)-t11.*t229.*1.82e-2-t11.*t232.*1.82e-2+t11.*t233.*1.82e-2-t11.*t266.*1.82e-2+t6.*t279.*9.1e-3+t11.*t298.*1.82e-2+t11.*t431.*1.82e-2-t11.*t442.*1.82e-2+t11.*t443.*1.82e-2+t11.*t503.*1.82e-2-t11.*t562.*1.82e-2+dq1.*dq6.*t6.*1.82e-2+t6.*t8.*t34.*1.56e-2-t3.*t6.*t42.*1.56e-2-t6.*t8.*t65.*3.12e-2+t3.*t4.*t75.*9.1e-3;
et13 = t11.*t23.*t50.*(-3.64e-2)-t11.*t24.*t50.*3.64e-2+t4.*t6.*t86-t6.*t23.*t68.*1.82e-2+t6.*t9.*t84+t10.*t11.*t79.*1.56e-2-t5.*t11.*t91.*3.12e-2-t3.*t6.*t100.*1.56e-2-t6.*t8.*t113.*3.12e-2+t8.*t11.*t114.*3.64e-2-t11.*t24.*t116.*3.64e-2+t6.*t8.*t140.*1.82e-2+t11.*t23.*t123.*1.82e-2+t8.*t11.*t139.*3.12e-2-t11.*t24.*t127.*3.64e-2-t3.*t4.*t166.*9.1e-3-t3.*t4.*t167.*9.1e-3;
et14 = t3.*t4.*t168.*9.1e-3-t10.*t11.*t177.*1.56e-2+t6.*t23.*t190.*1.82e-2+t6.*t8.*t210.*3.12e-2-t8.*t11.*t228.*3.64e-2+dq1.*dq2.*t6.*t9.*3.12e-2+dq4.*dq6.*t6.*t8.*1.82e-2-dq1.*dq6.*t6.*t24.*1.82e-2+ddq3.*t3.*t4.*t6-ddq6.*t3.*t4.*t11.*1.56e-2-ddq6.*t8.*t10.*t11.*9.1e-3-q3.*t6.*t8.*t34+q3.*t3.*t6.*t42+q3.*t6.*t8.*t65.*2.0-q3.*t10.*t11.*t79+q3.*t5.*t11.*t91.*2.0+q3.*t3.*t6.*t100+q3.*t10.*t11.*t102+q3.*t6.*t8.*t113.*2.0-q3.*t8.*t11.*t139.*2.0+q3.*t10.*t11.*t177-q3.*t6.*t8.*t210.*2.0;
et15 = q3.*t10.*t11.*t302+t3.*t4.*t6.*t13.*1.56e-2-t3.*t4.*t6.*t16.*1.56e-2-t6.*t8.*t10.*t16.*9.1e-3+t3.*t9.*t11.*t37.*1.56e-2+t3.*t4.*t11.*t43.*1.56e-2+t3.*t4.*t11.*t51.*3.12e-2+t3.*t6.*t9.*t53.*3.12e-2+t5.*t8.*t11.*t48.*(3.9e+1./6.25e+2)+t3.*t9.*t11.*t55.*1.56e-2-t3.*t9.*t11.*t56.*1.56e-2+t8.*t10.*t11.*t51.*3.64e-2+t8.*t11.*t23.*t48.*3.64e-2-t8.*t11.*t24.*t48.*3.64e-2+t11.*t23.*t24.*t50.*3.64e-2+t9.*t10.*t11.*t86;
et16 = t5.*t6.*t8.*t113.*1.82e-2-t3.*t6.*t10.*t118.*1.82e-2+t5.*t8.*t11.*t114.*3.12e-2-t3.*t6.*t10.*t126.*1.82e-2-t3.*t9.*t11.*t122.*1.82e-2-t5.*t6.*t8.*t129.*1.82e-2-t8.*t11.*t24.*t114.*7.28e-2+t4.*t10.*t11.*t163-t5.*t6.*t8.*t210.*3.64e-2+t8.*t10.*t11.*t208.*3.64e-2-dq1.*dq2.*q3.*t6.*t9.*2.0-dq1.*dq2.*t5.*t6.*t9.*1.82e-2-dq2.*dq3.*t4.*t6.*t8.*2.0-dq1.*dq2.*t4.*t10.*t11.*3.12e-2-dq5.*dq6.*t3.*t6.*t9.*1.82e-2;
et17 = dq1.*dq5.*t5.*t10.*t11.*3.64e-2+dq4.*dq6.*t3.*t9.*t11.*3.12e-2-dq1.*dq2.*t6.*t9.*t22.*(3.9e+1./6.25e+2)-dq1.*dq6.*t5.*t6.*t22.*3.12e-2+dq1.*dq3.*t5.*t11.*t22.*2.0-dq1.*dq4.*t6.*t10.*t22.*1.82e-2-dq4.*dq6.*t6.*t8.*t24.*1.82e-2+dq1.*dq5.*t10.*t11.*t22.*3.12e-2-dq1.*dq6.*t6.*t22.*t23.*1.82e-2+dq1.*dq6.*t6.*t22.*t24.*1.82e-2+ddq6.*q3.*t3.*t4.*t11+ddq6.*t3.*t6.*t9.*t10.*1.56e-2+ddq3.*t3.*t9.*t10.*t11+g.*t3.*t5.*t7.*t11-q3.*t3.*t4.*t6.*t13+q3.*t3.*t4.*t6.*t16-q3.*t3.*t4.*t11.*t51.*2.0-q3.*t3.*t6.*t9.*t53.*2.0;
et18 = q3.*t5.*t8.*t11.*t48.*-4.0-q3.*t3.*t9.*t11.*t55+q3.*t3.*t9.*t11.*t56+q3.*t3.*t4.*t11.*t87+q3.*t3.*t9.*t11.*t85-q3.*t5.*t8.*t11.*t114.*2.0-t3.*t9.*t10.*t11.*t16.*1.56e-2+t3.*t4.*t6.*t10.*t45.*3.64e-2-t8.*t9.*t10.*t11.*t49.*3.12e-2-t8.*t11.*t23.*t24.*t48.*3.64e-2+t4.*t6.*t9.*t10.*t91.*1.82e-2-t4.*t6.*t8.*t9.*t119.*3.64e-2-t3.*t4.*t5.*t11.*t128.*3.64e-2-ddq6.*q3.*t3.*t6.*t9.*t10+q3.*t3.*t9.*t10.*t11.*t16-dq4.*dq6.*q3.*t3.*t9.*t11.*2.0+dq1.*dq2.*q3.*t6.*t9.*t22.*4.0+dq1.*dq6.*q3.*t5.*t6.*t22.*2.0-dq1.*dq5.*q3.*t10.*t11.*t22.*2.0;
et19 = dq1.*dq3.*t3.*t6.*t8.*t9.*2.0-dq2.*dq6.*t3.*t4.*t6.*t9.*1.82e-2+dq1.*dq2.*t4.*t5.*t10.*t11.*3.64e-2+dq4.*dq6.*t3.*t4.*t6.*t10.*3.12e-2+dq2.*dq5.*t4.*t6.*t8.*t10.*1.82e-2+dq1.*dq6.*t3.*t8.*t9.*t11.*3.12e-2-dq2.*dq3.*t8.*t9.*t10.*t11.*2.0-dq2.*dq5.*t3.*t5.*t6.*t23.*1.82e-2+dq1.*dq2.*t5.*t6.*t9.*t22.*3.64e-2+dq1.*dq2.*t4.*t10.*t11.*t22.*(3.9e+1./6.25e+2)+dq1.*dq4.*t4.*t9.*t11.*t22.*3.64e-2-dq1.*dq5.*t5.*t10.*t11.*t22.*3.64e-2+dq1.*dq4.*t6.*t10.*t22.*t23.*3.64e-2+dq1.*dq6.*t6.*t22.*t23.*t24.*1.82e-2;
et20 = dq4.*dq6.*q3.*t3.*t4.*t6.*t10.*-2.0-dq1.*dq6.*q3.*t3.*t8.*t9.*t11.*2.0-dq1.*dq2.*q3.*t4.*t10.*t11.*t22.*4.0-dq1.*dq3.*t3.*t4.*t8.*t10.*t11.*2.0+dq1.*dq5.*t4.*t5.*t6.*t9.*t22.*1.82e-2+dq2.*dq6.*t3.*t4.*t6.*t9.*t24.*1.82e-2-dq1.*dq2.*t4.*t5.*t10.*t11.*t22.*7.28e-2-dq1.*dq6.*t4.*t9.*t10.*t11.*t22.*1.82e-2-dq1.*dq4.*t4.*t9.*t11.*t22.*t24.*3.64e-2-dq1.*dq5.*t5.*t10.*t11.*t22.*t23.*3.64e-2;
et21 = t3.*t62.*1.56e-2+t8.*t70.*1.56e-2-t3.*t82.*1.56e-2+t10.*t91.*3.12e-2-t10.*t116.*3.12e-2-t8.*t119.*(3.9e+1./6.25e+2)+t8.*t136.*3.12e-2-t5.*t177.*1.56e-2-t3.*t180.*1.56e-2-t8.*t208.*3.12e-2-t8.*t209.*3.12e-2-q3.*t3.*t62-q3.*t8.*t70+q3.*t3.*t82-q3.*t10.*t91.*2.0+q3.*t5.*t102+q3.*t10.*t116.*2.0+q3.*t8.*t119.*4.0-q3.*t8.*t136.*2.0+q3.*t5.*t177+q3.*t3.*t180+q3.*t8.*t208.*2.0+q3.*t8.*t209.*2.0+t5.*t9.*t86+t3.*t9.*t99.*1.56e-2+t4.*t5.*t163;
et22 = dq1.*dq2.*t4.*t5.*(-3.12e-2)+dq1.*dq5.*t5.*t22.*3.12e-2-dq1.*dq3.*t10.*t22.*2.0+ddq3.*t3.*t5.*t9-g.*t3.*t7.*t10-q3.*t3.*t9.*t99-dq1.*dq5.*q3.*t5.*t22.*2.0-dq2.*dq3.*t5.*t8.*t9.*2.0+dq1.*dq2.*t4.*t5.*t22.*(3.9e+1./6.25e+2)-dq1.*dq2.*q3.*t4.*t5.*t22.*4.0-dq1.*dq3.*t3.*t4.*t5.*t8.*2.0;
et23 = t10.*t79.*1.56e-2-t5.*t91.*3.12e-2+t8.*t139.*3.12e-2-t10.*t177.*1.56e-2-q3.*t10.*t79+q3.*t5.*t91.*2.0+q3.*t10.*t102-q3.*t8.*t139.*2.0+q3.*t10.*t177+q3.*t10.*t302+t3.*t9.*t37.*1.56e-2+t3.*t4.*t43.*1.56e-2+t3.*t4.*t51.*3.12e-2+t5.*t8.*t48.*(3.9e+1./6.25e+2)+t3.*t9.*t55.*1.56e-2-t3.*t9.*t56.*1.56e-2+t9.*t10.*t86+t5.*t8.*t114.*3.12e-2+t4.*t10.*t163-dq1.*dq2.*t4.*t10.*3.12e-2+dq1.*dq3.*t5.*t22.*2.0+dq1.*dq5.*t10.*t22.*3.12e-2+ddq3.*t3.*t9.*t10+g.*t3.*t5.*t7;
et24 = q3.*t3.*t4.*t51.*-2.0-q3.*t5.*t8.*t48.*4.0-q3.*t3.*t9.*t55+q3.*t3.*t9.*t56+q3.*t3.*t4.*t87+q3.*t3.*t9.*t85-q3.*t5.*t8.*t114.*2.0-t8.*t9.*t10.*t49.*3.12e-2-dq1.*dq5.*q3.*t10.*t22.*2.0-dq2.*dq3.*t8.*t9.*t10.*2.0+dq1.*dq2.*t4.*t10.*t22.*(3.9e+1./6.25e+2)-dq1.*dq2.*q3.*t4.*t10.*t22.*4.0-dq1.*dq3.*t3.*t4.*t8.*t10.*2.0;
et25 = t68-t73-t144+t145-t146-t186-t190+t191-t257-t278+t279+t309+t325-t338-t356+t390+t433+t453-t464+t482+t489+t522+t551-t25.*t68.*2.0+t25.*t73.*2.0+t25.*t144.*2.0-t25.*t145.*2.0+t25.*t146.*2.0+t25.*t190.*2.0-t25.*t191.*2.0+t25.*t278.*2.0-t25.*t279.*2.0+t25.*t280.*2.0+dq1.*dq6.*t22.*2.0-dq1.*dq6.*t24.*2.0-t6.*t11.*t50.*4.0+t6.*t11.*t71.*2.0-t6.*t11.*t91.*2.0+t6.*t11.*t92.*2.0+t23.*t25.*t68.*4.0-t3.*t10.*t118.*2.0+t6.*t11.*t123.*4.0-t6.*t11.*t124.*4.0-t5.*t8.*t129.*2.0-t6.*t11.*t127.*4.0+t6.*t11.*t142.*4.0-t8.*t25.*t140.*4.0+t6.*t11.*t173.*2.0+t3.*t4.*t195-t5.*t8.*t210.*4.0-t6.*t11.*t213.*4.0;
et26 = t6.*t11.*t214.*4.0-t6.*t11.*t215.*4.0-t23.*t25.*t190.*4.0+t6.*t11.*t229.*2.0+t6.*t11.*t232.*4.0-t6.*t11.*t233.*2.0+t6.*t11.*t266.*2.0-t6.*t11.*t298.*4.0-t6.*t11.*t431.*2.0-t6.*t11.*t443.*2.0-t6.*t11.*t503.*2.0+t6.*t11.*t562.*2.0-dq5.*dq6.*t3.*t9.*2.0-dq4.*dq6.*t8.*t24.*2.0-dq1.*dq6.*t22.*t23.*4.0+dq1.*dq6.*t22.*t24.*2.0-dq1.*dq6.*t22.*t25.*4.0+dq1.*dq6.*t24.*t25.*4.0+t6.*t8.*t11.*t48.*4.0+t6.*t11.*t23.*t50.*8.0+t6.*t11.*t24.*t50.*4.0-t6.*t8.*t11.*t114.*4.0-t4.*t8.*t9.*t119.*4.0-t5.*t8.*t25.*t113.*4.0+t3.*t10.*t25.*t118.*4.0+t6.*t11.*t24.*t116.*4.0-t6.*t11.*t23.*t123.*8.0+t3.*t10.*t25.*t126.*4.0+t5.*t8.*t25.*t129.*4.0+t6.*t11.*t24.*t127.*4.0+t5.*t8.*t25.*t210.*8.0+t6.*t8.*t11.*t228.*4.0;
et27 = t4.*t9.*t10.*t234.*-4.0+t3.*t5.*t9.*t300.*2.0-dq2.*dq6.*t3.*t4.*t9.*4.0+dq1.*dq2.*t5.*t9.*t25.*4.0+dq5.*dq6.*t3.*t9.*t25.*4.0+dq1.*dq4.*t10.*t22.*t25.*4.0+dq4.*dq6.*t8.*t24.*t25.*4.0+dq1.*dq6.*t22.*t23.*t24.*2.0+dq1.*dq6.*t22.*t23.*t25.*8.0-dq1.*dq6.*t22.*t24.*t25.*4.0-t6.*t8.*t10.*t11.*t51.*4.0-t3.*t4.*t10.*t25.*t45.*8.0-t6.*t8.*t11.*t23.*t48.*8.0+t6.*t8.*t11.*t24.*t48.*4.0-t6.*t11.*t23.*t24.*t50.*4.0+t3.*t6.*t9.*t11.*t122.*8.0+t6.*t8.*t11.*t24.*t114.*8.0+t4.*t8.*t9.*t25.*t119.*8.0-t6.*t8.*t10.*t11.*t208.*4.0+t6.*t8.*t11.*t23.*t24.*t48.*4.0+t3.*t4.*t5.*t6.*t11.*t128.*4.0-dq1.*dq5.*t5.*t6.*t10.*t11.*4.0+dq2.*dq6.*t3.*t4.*t9.*t24.*2.0+dq2.*dq6.*t3.*t4.*t9.*t25.*8.0-dq2.*dq5.*t4.*t8.*t10.*t25.*4.0;
et28 = dq2.*dq5.*t3.*t5.*t23.*t25.*4.0-dq1.*dq2.*t5.*t9.*t22.*t25.*8.0-dq1.*dq4.*t10.*t22.*t23.*t25.*8.0-dq1.*dq6.*t22.*t23.*t24.*t25.*4.0-dq1.*dq2.*t4.*t5.*t6.*t10.*t11.*4.0-dq1.*dq4.*t4.*t6.*t9.*t11.*t22.*8.0+dq1.*dq5.*t5.*t6.*t10.*t11.*t22.*4.0-dq1.*dq5.*t4.*t5.*t9.*t22.*t25.*4.0-dq2.*dq6.*t3.*t4.*t9.*t24.*t25.*4.0+dq1.*dq2.*t4.*t5.*t6.*t10.*t11.*t22.*8.0+dq1.*dq6.*t4.*t6.*t9.*t10.*t11.*t22.*8.0+dq1.*dq4.*t4.*t6.*t9.*t11.*t22.*t24.*4.0+dq1.*dq5.*t5.*t6.*t10.*t11.*t22.*t23.*4.0;
et29 = -t11.*t60+t8.*t75-t11.*t79+t11.*t102-t8.*t143.*2.0+t8.*t160+t8.*t168-t11.*t174+t11.*t177+t8.*t251.*2.0+t8.*t272+t11.*t302+t8.*t313+t8.*t336+dq1.*dq5.*t11.*2.0-t5.*t6.*t33+t5.*t6.*t54+t11.*t24.*t60.*2.0+t11.*t24.*t79.*2.0+t8.*t24.*t143.*4.0+t11.*t24.*t174.*2.0-t11.*t24.*t177.*2.0+dq4.*dq5.*t8.*t11.*2.0-dq1.*dq5.*t11.*t22.*2.0-dq1.*dq5.*t11.*t24.*4.0-ddq6.*t3.*t6.*t9-ddq1.*t5.*t10.*t11.*2.0+t3.*t9.*t11.*t16+t3.*t5.*t6.*t36+t3.*t6.*t10.*t42-t3.*t4.*t11.*t46.*2.0-t8.*t10.*t11.*t35.*2.0+t5.*t6.*t23.*t33.*2.0-t3.*t4.*t6.*t55-t3.*t4.*t6.*t56-t5.*t10.*t11.*t50.*4.0-t6.*t8.*t10.*t52.*2.0-t5.*t6.*t23.*t54.*2.0;
et30 = t5.*t10.*t11.*t91.*2.0+t3.*t6.*t10.*t100+t6.*t8.*t10.*t113.*2.0+t3.*t6.*t9.*t120.*2.0-t5.*t8.*t11.*t119.*4.0-t8.*t9.*t11.*t121.*2.0-t5.*t10.*t11.*t127.*4.0-t5.*t8.*t11.*t209.*8.0+t5.*t10.*t11.*t232.*2.0+t5.*t6.*t8.*t289-dq4.*dq6.*t3.*t4.*t6.*2.0+dq2.*dq6.*t3.*t5.*t11.*2.0-dq1.*dq2.*t6.*t9.*t10.*2.0-dq1.*dq6.*t5.*t6.*t10.*2.0+dq1.*dq4.*t5.*t6.*t22.*2.0-dq1.*dq2.*t4.*t11.*t22.*4.0-dq1.*dq2.*t4.*t11.*t24.*4.0-dq4.*dq5.*t8.*t11.*t24.*4.0-dq1.*dq5.*t11.*t22.*t23.*2.0+dq1.*dq5.*t11.*t22.*t24.*4.0+ddq6.*t3.*t4.*t10.*t11+t3.*t4.*t6.*t10.*t16-t3.*t4.*t5.*t6.*t45.*4.0-t3.*t4.*t10.*t11.*t51.*4.0+t3.*t4.*t11.*t24.*t46.*4.0+t4.*t5.*t9.*t11.*t68.*2.0+t5.*t10.*t11.*t23.*t50.*4.0-t8.*t9.*t11.*t24.*t49.*4.0;
et31 = t4.*t5.*t6.*t9.*t91.*-2.0+t3.*t6.*t9.*t10.*t117.*2.0-t5.*t8.*t11.*t23.*t119.*4.0-t4.*t5.*t9.*t11.*t190.*2.0-dq1.*dq6.*t3.*t4.*t6.*t8.*2.0-dq4.*dq6.*t3.*t9.*t10.*t11.*2.0+dq4.*dq6.*t3.*t4.*t6.*t24.*2.0-dq2.*dq5.*t3.*t6.*t10.*t23.*2.0+dq1.*dq2.*t6.*t9.*t10.*t22.*4.0+dq1.*dq6.*t5.*t6.*t10.*t22.*2.0-dq2.*dq6.*t3.*t5.*t11.*t23.*2.0+dq2.*dq6.*t6.*t8.*t9.*t24.*2.0-dq1.*dq4.*t5.*t6.*t22.*t23.*4.0+dq1.*dq2.*t4.*t11.*t22.*t24.*8.0+dq1.*dq5.*t11.*t22.*t23.*t24.*4.0+dq1.*dq6.*t3.*t4.*t6.*t8.*t24.*4.0+dq1.*dq5.*t4.*t6.*t9.*t10.*t22.*2.0+dq1.*dq6.*t4.*t5.*t9.*t11.*t22.*2.0+dq1.*dq6.*t5.*t6.*t10.*t22.*t23.*2.0-dq1.*dq4.*t4.*t5.*t9.*t10.*t11.*t22.*4.0;
et32 = -t6.*t60+t8.*t63-t8.*t72+t8.*t83+t6.*t102-t8.*t137.*2.0+t8.*t153-t6.*t174+t6.*t177+t8.*t181-t8.*t265.*2.0+t8.*t293+t6.*t302+t8.*t317+dq1.*dq5.*t6.*2.0+t5.*t11.*t33-t5.*t11.*t54+t6.*t24.*t60.*2.0+t8.*t24.*t72.*2.0+t8.*t24.*t137.*4.0+t6.*t24.*t174.*2.0-t6.*t24.*t177.*2.0+dq4.*dq5.*t6.*t8.*2.0-dq1.*dq5.*t6.*t22.*2.0-dq1.*dq5.*t6.*t24.*4.0-ddq1.*t5.*t6.*t10.*2.0+ddq6.*t3.*t9.*t11+t3.*t6.*t9.*t16-t3.*t5.*t11.*t36-t3.*t4.*t6.*t46.*2.0-t6.*t8.*t10.*t35.*2.0-t3.*t10.*t11.*t42-t5.*t6.*t10.*t50.*4.0-t5.*t11.*t23.*t33.*2.0+t3.*t4.*t11.*t55+t3.*t4.*t11.*t56+t8.*t10.*t11.*t52.*2.0+t5.*t11.*t23.*t54.*2.0+t5.*t6.*t10.*t91.*2.0;
et33 = -t3.*t10.*t11.*t100-t5.*t6.*t8.*t119.*4.0-t8.*t10.*t11.*t113.*2.0-t3.*t9.*t11.*t120.*2.0-t6.*t8.*t9.*t121.*2.0-t5.*t6.*t10.*t127.*4.0-t5.*t6.*t8.*t209.*8.0+t5.*t6.*t10.*t232.*2.0+dq2.*dq6.*t3.*t5.*t6.*2.0+dq4.*dq6.*t3.*t4.*t11.*2.0+dq1.*dq2.*t9.*t10.*t11.*2.0+dq1.*dq6.*t5.*t10.*t11.*2.0-dq1.*dq2.*t4.*t6.*t22.*4.0-dq1.*dq2.*t4.*t6.*t24.*4.0-dq1.*dq4.*t5.*t11.*t22.*2.0-dq4.*dq5.*t6.*t8.*t24.*4.0-dq1.*dq5.*t6.*t22.*t23.*2.0+dq1.*dq5.*t6.*t22.*t24.*4.0+ddq6.*t3.*t4.*t6.*t10-t3.*t4.*t10.*t11.*t16+t3.*t4.*t5.*t11.*t45.*4.0-t3.*t4.*t6.*t10.*t51.*4.0+t3.*t4.*t6.*t24.*t46.*4.0+t4.*t5.*t6.*t9.*t68.*2.0+t5.*t6.*t10.*t23.*t50.*4.0-t6.*t8.*t9.*t24.*t49.*4.0+t4.*t5.*t9.*t11.*t91.*2.0;
et34 = t3.*t9.*t10.*t11.*t117.*-2.0-t5.*t6.*t8.*t23.*t119.*4.0-t4.*t5.*t6.*t9.*t190.*2.0-t4.*t5.*t8.*t9.*t11.*t48.*4.0+dq1.*dq6.*t3.*t4.*t8.*t11.*2.0-dq4.*dq6.*t3.*t6.*t9.*t10.*2.0-dq2.*dq6.*t3.*t5.*t6.*t23.*2.0-dq4.*dq6.*t3.*t4.*t11.*t24.*2.0+dq2.*dq5.*t3.*t10.*t11.*t23.*2.0-dq1.*dq2.*t9.*t10.*t11.*t22.*4.0-dq1.*dq6.*t5.*t10.*t11.*t22.*2.0+dq1.*dq2.*t4.*t6.*t22.*t24.*8.0-dq2.*dq6.*t8.*t9.*t11.*t24.*2.0+dq1.*dq4.*t5.*t11.*t22.*t23.*4.0+dq1.*dq5.*t6.*t22.*t23.*t24.*4.0+dq1.*dq6.*t4.*t5.*t6.*t9.*t22.*2.0-dq1.*dq6.*t3.*t4.*t8.*t11.*t24.*4.0-dq1.*dq5.*t4.*t9.*t10.*t11.*t22.*2.0-dq1.*dq6.*t5.*t10.*t11.*t22.*t23.*2.0-dq1.*dq4.*t4.*t5.*t6.*t9.*t10.*t22.*4.0;
et35 = -t60-t79+t102-t174+t177-t200-t242+t302+dq1.*dq5.*2.0-ddq1.*t28+t24.*t60.*2.0+t24.*t79.*2.0+t24.*t174.*2.0-t24.*t177.*2.0+dq4.*dq5.*t8.*2.0-dq1.*dq5.*t22.*2.0-dq1.*dq5.*t24.*4.0-t3.*t4.*t46.*2.0-t8.*t10.*t35.*2.0-t5.*t10.*t50.*4.0+t8.*t24.*t59.*4.0+t5.*t10.*t91.*2.0-t5.*t8.*t119.*4.0-t5.*t10.*t127.*4.0-t5.*t8.*t209.*8.0+t5.*t10.*t232.*2.0-dq1.*dq2.*t4.*t24.*4.0-dq4.*dq5.*t8.*t24.*4.0-dq1.*dq5.*t22.*t23.*2.0+dq1.*dq5.*t22.*t24.*4.0-t3.*t4.*t10.*t51.*4.0+t3.*t4.*t24.*t46.*4.0+t4.*t5.*t9.*t68.*2.0+t5.*t10.*t23.*t50.*4.0-t8.*t9.*t24.*t49.*4.0-t5.*t8.*t23.*t119.*4.0-t4.*t5.*t9.*t190.*2.0+dq1.*dq2.*t4.*t22.*t24.*8.0;
et36 = dq1.*dq5.*t22.*t23.*t24.*4.0-dq1.*dq4.*t4.*t5.*t9.*t10.*t22.*4.0;
et37 = t92-t107+t123-t127+t133+t142+t173+t214+t217+t223+t229+t232+t234+t244+t246+t247-t254+t255+t266-t288-t311+t342+t344+t357+t364-t365+t366+t385+t391-t395-t398-t400+t401+t404+t405+t412+t413+t442-t443+t449+t454+t459+t462-t463+t469+t473+t477+t479-t487+t500-t501+t502+t504-t512+t518+t521-t531+t548+t549+t550+t553+t558-t559+t560+t562+t564+t566+t570+t573-t575+t578+t588+t598+t608+t610+t611+t613+t614+t619+t621+t631+t633+t636+t639-t640+t641-t645-t658+t661-t664+t665+t666+t669+t679+t25.*t159+t24.*t192+t25.*t193+t24.*t270+t25.*t315-t8.*t362.*2.0+t24.*t419+t25.*t418+t25.*t424+t25.*t478-t8.*t498.*2.0+t25.*t585+t25.*t647;
et38 = t25.*t652+t25.*t653+t25.*t654-t8.*t25.*t48.*2.0-t23.*t24.*t50.*2.0-t24.*t25.*t50.*2.0-t24.*t25.*t116.*2.0-t24.*t25.*t127.*2.0-t8.*t24.*t25.*t114.*4.0-dq1.*dq2.*t4.*t5.*t10.*2.0-t5.*t6.*t8.*t11.*t113.*2.0-t3.*t4.*t5.*t25.*t128.*2.0-t3.*t4.*t6.*t10.*t11.*t45.*4.0-t4.*t6.*t9.*t10.*t11.*t91.*2.0-dq1.*dq5.*t5.*t10.*t22.*t25.*2.0-dq1.*dq6.*t6.*t11.*t22.*t24.*2.0-dq2.*dq5.*t4.*t6.*t8.*t10.*t11.*2.0-dq1.*dq2.*t5.*t6.*t9.*t11.*t22.*4.0-dq1.*dq4.*t6.*t10.*t11.*t22.*t23.*4.0-dq1.*dq6.*t6.*t11.*t22.*t23.*t24.*2.0-dq1.*dq5.*t4.*t5.*t6.*t9.*t11.*t22.*2.0-dq2.*dq6.*t3.*t4.*t6.*t9.*t11.*t24.*2.0;
et39 = t50+t91+t124+t127+t159+t203+t213+t215+t217+t222+t236-t247+t254-t255+t270+t283+t298+t323+t343-t364+t365-t366+t368+t384+t386+t388+t395+t398+t400-t401-t404-t405-t413+t419-t449-t459-t462+t463+t487+t499-t500+t501+t511+t512-t521+t527+t536-t558+t559-t560-t564+t575-t578+t587-t588+t593+t595-t598+t609-t614+t615+t618-t619-t621+t625+t628+t640-t641+t644+t645+t648+t655+t658+t659+t660-t661+t662+t663+t664+t674+t675+t677+t690+t691+t692+t693+t25.*t192-t8.*t25.*t114.*2.0+t24.*t25.*t192+t24.*t25.*t270+t24.*t25.*t419-t8.*t10.*t25.*t51.*2.0-t8.*t23.*t25.*t48.*4.0-t23.*t24.*t25.*t50.*2.0;
et40 = t8.*t10.*t25.*t208.*-2.0+t3.*t4.*t11.*t313-t3.*t6.*t10.*t11.*t126.*2.0-t5.*t6.*t8.*t11.*t129.*2.0-t4.*t6.*t8.*t9.*t11.*t119.*4.0-dq1.*dq2.*t5.*t6.*t9.*t11.*2.0-dq1.*dq2.*t4.*t5.*t10.*t25.*2.0-dq1.*dq4.*t6.*t10.*t11.*t22.*2.0-dq4.*dq6.*t6.*t8.*t11.*t24.*2.0-dq2.*dq5.*t3.*t5.*t6.*t11.*t23.*2.0;
et41 = t6.*t36.*1.82e-2+t9.*t63.*9.1e-3+t11.*t62.*9.1e-3-t11.*t66.*9.1e-3+t11.*t82.*9.1e-3+t6.*t93.*1.82e-2+t6.*t94.*1.82e-2+t6.*t118.*1.82e-2-t9.*t137.*1.82e-2+t11.*t141.*9.1e-3-t6.*t154.*1.82e-2+t9.*t153.*1.82e-2-t11.*t175.*9.1e-3-t11.*t179.*9.1e-3-t9.*t182.*9.1e-3+t11.*t180.*9.1e-3;
et42 = t6.*t198.*(-3.64e-2)+t6.*t212.*1.82e-2-t6.*t235.*1.82e-2-t6.*t264.*1.82e-2-t6.*t285.*1.82e-2-t6.*t287.*1.82e-2-t6.*t369.*1.82e-2+t6.*t370.*1.82e-2+t9.*t374.*1.82e-2-t9.*t529.*1.82e-2+t6.*t599.*1.82e-2-ddq2.*t5.*t6.*3.12e-2-ddq4.*t4.*t11.*1.56e-2-ddq6.*t6.*t9.*1.56e-2-ddq3.*t9.*t11+t9.*t11.*t12.*1.56e-2+t9.*t11.*t14.*1.56e-2;
et43 = t9.*t11.*t16.*1.56e-2-t5.*t6.*t36.*1.56e-2-t4.*t11.*t39.*1.56e-2-t4.*t6.*t45.*3.64e-2+t5.*t6.*t47.*3.12e-2+t6.*t10.*t42.*1.56e-2+t4.*t6.*t56.*1.56e-2+t4.*t11.*t53.*3.12e-2-t6.*t24.*t47.*3.64e-2+t9.*t11.*t64+t5.*t6.*t76+t6.*t10.*t77.*1.56e-2+t11.*t23.*t66.*1.82e-2+t6.*t10.*t98.*1.56e-2+t6.*t10.*t100.*1.56e-2+t6.*t9.*t120.*3.12e-2+t4.*t6.*t129.*1.82e-2+t6.*t23.*t121.*1.82e-2;
et44 = t6.*t24.*t126.*(-3.64e-2)-t9.*t11.*t150.*3.12e-2+t9.*t24.*t137.*1.82e-2+t6.*t24.*t198.*3.64e-2+t6.*t22.*t285.*3.64e-2+dq2.*dq3.*t5.*t6.*2.0-dq4.*dq6.*t4.*t6.*3.12e-2+dq2.*dq5.*t6.*t10.*3.12e-2+dq2.*dq6.*t5.*t11.*3.12e-2-dq5.*dq6.*t4.*t11.*1.82e-2-dq2.*dq4.*t10.*t11.*1.82e-2-dq2.*dq6.*t11.*t23.*1.82e-2-dq2.*dq6.*t11.*t24.*1.82e-2+ddq2.*q3.*t5.*t6.*2.0+ddq4.*q3.*t4.*t11+ddq6.*q3.*t6.*t9-ddq3.*t4.*t6.*t10+ddq6.*t4.*t10.*t11.*1.56e-2;
et45 = -q3.*t9.*t11.*t14-q3.*t9.*t11.*t16+q3.*t5.*t6.*t36+q3.*t4.*t11.*t39-q3.*t5.*t6.*t47.*2.0-q3.*t6.*t10.*t42-q3.*t4.*t6.*t56-q3.*t4.*t11.*t53.*2.0+q3.*t9.*t11.*t58-q3.*t6.*t10.*t77-q3.*t6.*t10.*t100-q3.*t6.*t9.*t120.*2.0+q3.*t9.*t11.*t150.*2.0+q3.*t6.*t10.*t320+t4.*t6.*t10.*t16.*1.56e-2+t4.*t5.*t11.*t46.*1.82e-2+t4.*t6.*t24.*t45.*3.64e-2+t9.*t10.*t11.*t52.*1.82e-2+t4.*t6.*t10.*t64-t6.*t10.*t22.*t98.*3.12e-2-t9.*t10.*t11.*t113.*3.64e-2+t9.*t10.*t11.*t122.*1.82e-2-t5.*t6.*t9.*t209.*3.64e-2;
et46 = dq4.*dq6.*q3.*t4.*t6.*2.0-dq2.*dq5.*q3.*t6.*t10.*2.0-dq2.*dq6.*q3.*t5.*t11.*2.0-dq1.*dq5.*t3.*t5.*t11.*1.82e-2-dq1.*dq6.*t4.*t6.*t8.*3.12e-2-dq2.*dq5.*t5.*t6.*t10.*3.64e-2+dq1.*dq4.*t8.*t9.*t11.*3.12e-2-dq4.*dq6.*t9.*t10.*t11.*3.12e-2+dq2.*dq4.*t10.*t11.*t23.*3.64e-2+dq2.*dq6.*t11.*t23.*t24.*1.82e-2-ddq6.*q3.*t4.*t10.*t11-q3.*t4.*t6.*t10.*t16+q3.*t4.*t6.*t10.*t58-t3.*t5.*t6.*t8.*t12.*3.12e-2+q3.*t3.*t5.*t6.*t8.*t12.*2.0+dq1.*dq6.*q3.*t4.*t6.*t8.*2.0-dq1.*dq4.*q3.*t8.*t9.*t11.*2.0+dq4.*dq6.*q3.*t9.*t10.*t11.*2.0;
et47 = dq1.*dq4.*t4.*t6.*t8.*t10.*3.12e-2+dq1.*dq6.*t3.*t4.*t9.*t11.*1.82e-2-dq1.*dq4.*t5.*t8.*t9.*t11.*1.82e-2-dq1.*dq6.*t8.*t9.*t10.*t11.*3.12e-2+dq1.*dq5.*t3.*t5.*t11.*t23.*1.82e-2+dq2.*dq5.*t5.*t6.*t10.*t23.*3.64e-2-dq1.*dq4.*q3.*t4.*t6.*t8.*t10.*2.0+dq1.*dq6.*q3.*t8.*t9.*t10.*t11.*2.0-dq1.*dq4.*t4.*t5.*t6.*t8.*t10.*3.64e-2-dq1.*dq6.*t3.*t4.*t9.*t11.*t24.*1.82e-2;
et48 = t11.*t36.*1.82e-2-t6.*t62.*9.1e-3+t6.*t66.*9.1e-3-t9.*t74.*9.1e-3+t9.*t75.*9.1e-3+t11.*t93.*1.82e-2+t11.*t94.*1.82e-2+t11.*t118.*1.82e-2-t6.*t141.*9.1e-3-t11.*t138.*1.82e-2-t9.*t147.*1.82e-2-t11.*t154.*1.82e-2-t9.*t167.*9.1e-3+t9.*t168.*9.1e-3+t6.*t175.*9.1e-3+t6.*t179.*9.1e-3;
et49 = t11.*t198.*(-3.64e-2)+t11.*t212.*1.82e-2-t11.*t235.*1.82e-2-t11.*t264.*1.82e-2-t11.*t285.*1.82e-2-t11.*t287.*1.82e-2-t9.*t349.*1.82e-2-t11.*t369.*1.82e-2+t11.*t370.*1.82e-2+t11.*t430.*1.82e-2+t9.*t513.*1.82e-2+t11.*t599.*1.82e-2+ddq4.*t4.*t6.*1.56e-2-ddq2.*t5.*t11.*3.12e-2+ddq3.*t6.*t9-ddq6.*t9.*t11.*1.56e-2-t6.*t9.*t12.*1.56e-2;
et50 = t6.*t9.*t14.*(-1.56e-2)-t6.*t9.*t16.*1.56e-2+t4.*t6.*t39.*1.56e-2-t5.*t11.*t36.*1.56e-2-t4.*t11.*t45.*3.64e-2-t4.*t6.*t53.*3.12e-2+t5.*t11.*t47.*3.12e-2+t10.*t11.*t42.*1.56e-2+t4.*t11.*t56.*1.56e-2-t6.*t9.*t64-t11.*t24.*t47.*3.64e-2+t5.*t11.*t76-t6.*t23.*t66.*1.82e-2+t10.*t11.*t77.*1.56e-2+t10.*t11.*t98.*1.56e-2+t10.*t11.*t100.*1.56e-2+t9.*t11.*t120.*3.12e-2+t4.*t11.*t129.*1.82e-2;
et51 = t11.*t23.*t121.*1.82e-2-t11.*t24.*t126.*3.64e-2+t6.*t9.*t150.*3.12e-2+t11.*t24.*t198.*3.64e-2+t11.*t22.*t285.*3.64e-2-dq2.*dq6.*t5.*t6.*3.12e-2+dq2.*dq3.*t5.*t11.*2.0+dq5.*dq6.*t4.*t6.*1.82e-2+dq2.*dq4.*t6.*t10.*1.82e-2-dq4.*dq6.*t4.*t11.*3.12e-2+dq2.*dq5.*t10.*t11.*3.12e-2+dq2.*dq6.*t6.*t23.*1.82e-2+dq2.*dq6.*t6.*t24.*1.82e-2-ddq4.*q3.*t4.*t6+ddq2.*q3.*t5.*t11.*2.0+ddq6.*q3.*t9.*t11-ddq6.*t4.*t6.*t10.*1.56e-2-ddq3.*t4.*t10.*t11+q3.*t6.*t9.*t12;
et52 = q3.*t6.*t9.*t14+q3.*t6.*t9.*t16-q3.*t4.*t6.*t39+q3.*t5.*t11.*t36+q3.*t4.*t6.*t53.*2.0-q3.*t5.*t11.*t47.*2.0-q3.*t10.*t11.*t42-q3.*t4.*t11.*t56-q3.*t10.*t11.*t77-q3.*t10.*t11.*t100-q3.*t9.*t11.*t120.*2.0-q3.*t6.*t9.*t150.*2.0+q3.*t10.*t11.*t320+t4.*t10.*t11.*t16.*1.56e-2-t4.*t5.*t6.*t46.*1.82e-2-t6.*t9.*t10.*t52.*1.82e-2+t4.*t11.*t24.*t45.*3.64e-2+t4.*t10.*t11.*t64+t6.*t9.*t10.*t113.*3.64e-2-t10.*t11.*t22.*t98.*3.12e-2-t6.*t9.*t10.*t122.*1.82e-2-t5.*t9.*t11.*t209.*3.64e-2;
et53 = dq2.*dq6.*q3.*t5.*t6.*2.0+dq4.*dq6.*q3.*t4.*t11.*2.0-dq2.*dq5.*q3.*t10.*t11.*2.0+dq1.*dq5.*t3.*t5.*t6.*1.82e-2-dq1.*dq4.*t6.*t8.*t9.*3.12e-2-dq1.*dq6.*t4.*t8.*t11.*3.12e-2-dq2.*dq5.*t5.*t10.*t11.*3.64e-2+dq4.*dq6.*t6.*t9.*t10.*3.12e-2-dq2.*dq4.*t6.*t10.*t23.*3.64e-2-dq2.*dq6.*t6.*t23.*t24.*1.82e-2+ddq6.*q3.*t4.*t6.*t10-q3.*t4.*t10.*t11.*t16+q3.*t4.*t10.*t11.*t58-t3.*t5.*t8.*t11.*t12.*3.12e-2+q3.*t3.*t5.*t8.*t11.*t12.*2.0+dq1.*dq4.*q3.*t6.*t8.*t9.*2.0+dq1.*dq6.*q3.*t4.*t8.*t11.*2.0-dq4.*dq6.*q3.*t6.*t9.*t10.*2.0;
et54 = dq1.*dq6.*t3.*t4.*t6.*t9.*(-1.82e-2)+dq1.*dq4.*t5.*t6.*t8.*t9.*1.82e-2+dq1.*dq4.*t4.*t8.*t10.*t11.*3.12e-2+dq1.*dq6.*t6.*t8.*t9.*t10.*3.12e-2-dq1.*dq5.*t3.*t5.*t6.*t23.*1.82e-2+dq2.*dq5.*t5.*t10.*t11.*t23.*3.64e-2-dq1.*dq4.*q3.*t4.*t8.*t10.*t11.*2.0-dq1.*dq6.*q3.*t6.*t8.*t9.*t10.*2.0-dq1.*dq4.*t4.*t5.*t8.*t10.*t11.*3.64e-2+dq1.*dq6.*t3.*t4.*t6.*t9.*t24.*1.82e-2;
et55 = ddq2.*t10.*3.12e-2+t9.*t35.*1.56e-2+t10.*t36.*1.56e-2-t10.*t47.*3.12e-2+t9.*t67.*1.56e-2-t10.*t76+t5.*t98.*1.56e-2+t4.*t101.*1.56e-2+t5.*t100.*1.56e-2-t10.*t126.*3.12e-2+dq2.*dq5.*t5.*3.12e-2-dq2.*dq3.*t10.*2.0-ddq2.*q3.*t10.*2.0-ddq3.*t4.*t5-q3.*t9.*t35-q3.*t10.*t36+q3.*t10.*t47.*2.0-q3.*t9.*t67-q3.*t5.*t100+q3.*t10.*t126.*2.0+q3.*t4.*t195+q3.*t5.*t320+t4.*t5.*t64-t5.*t22.*t98.*3.12e-2-dq2.*dq5.*q3.*t5.*2.0+q3.*t4.*t5.*t58;
et56 = t3.*t8.*t10.*t12.*3.12e-2+dq1.*dq4.*t4.*t5.*t8.*3.12e-2-q3.*t3.*t8.*t10.*t12.*2.0-dq1.*dq4.*q3.*t4.*t5.*t8.*2.0;
et57 = ddq2.*t5.*(-3.12e-2)-t5.*t36.*1.56e-2+t5.*t47.*3.12e-2+t10.*t42.*1.56e-2+t4.*t56.*1.56e-2+t5.*t76+t10.*t77.*1.56e-2+t10.*t98.*1.56e-2+t10.*t100.*1.56e-2+t9.*t120.*3.12e-2+dq2.*dq3.*t5.*2.0+dq2.*dq5.*t10.*3.12e-2+ddq2.*q3.*t5.*2.0-ddq3.*t4.*t10+q3.*t5.*t36-q3.*t5.*t47.*2.0-q3.*t10.*t42-q3.*t4.*t56-q3.*t10.*t77-q3.*t10.*t100-q3.*t9.*t120.*2.0+q3.*t10.*t320+t4.*t10.*t64-t10.*t22.*t98.*3.12e-2-dq2.*dq5.*q3.*t10.*2.0+q3.*t4.*t10.*t58;
et58 = t3.*t5.*t8.*t12.*(-3.12e-2)+dq1.*dq4.*t4.*t8.*t10.*3.12e-2+q3.*t3.*t5.*t8.*t12.*2.0-dq1.*dq4.*q3.*t4.*t8.*t10.*2.0;
et59 = t57-t62+t66-t82-t141+t170+t175+t179-t180-t202-t261-t292+t305-t337+t451-t474+t582-dq2.*dq6.*2.0+ddq2.*t29+t25.*t62.*2.0-t25.*t66.*2.0+t25.*t82.*2.0+t25.*t141.*2.0-t25.*t175.*2.0-t25.*t179.*2.0+t25.*t180.*2.0+dq5.*dq6.*t4.*2.0+dq2.*dq6.*t23.*4.0+dq2.*dq6.*t24.*2.0+dq2.*dq6.*t25.*4.0-t6.*t11.*t36.*2.0-t6.*t11.*t49.*4.0-t9.*t10.*t52.*2.0+t9.*t25.*t69.*4.0-t6.*t11.*t93.*4.0-t6.*t11.*t94.*2.0+t23.*t25.*t66.*4.0-t6.*t11.*t118.*4.0+t6.*t11.*t121.*4.0-t9.*t10.*t122.*2.0-t6.*t11.*t130.*4.0+t9.*t11.*t137.*4.0+t9.*t10.*t148.*2.0+t6.*t11.*t198.*8.0-t6.*t11.*t212.*4.0+t6.*t11.*t235.*2.0+t9.*t10.*t253.*2.0;
et60 = t9.*t25.*t239.*4.0+t6.*t11.*t285.*2.0+t6.*t11.*t287.*2.0+t6.*t11.*t369.*4.0-t6.*t11.*t370.*2.0-t9.*t25.*t439.*4.0-t6.*t11.*t599.*2.0-dq5.*dq6.*t4.*t25.*4.0-dq2.*dq4.*t10.*t25.*4.0-dq2.*dq6.*t23.*t24.*2.0-dq2.*dq6.*t23.*t25.*8.0-dq2.*dq6.*t24.*t25.*4.0+t4.*t6.*t11.*t45.*8.0+t4.*t5.*t25.*t46.*4.0+t6.*t11.*t24.*t47.*4.0+t9.*t10.*t25.*t52.*4.0-t4.*t6.*t11.*t129.*8.0-t9.*t10.*t25.*t113.*8.0-t6.*t11.*t23.*t121.*8.0+t9.*t10.*t25.*t122.*4.0+t6.*t11.*t24.*t126.*4.0-t9.*t11.*t24.*t137.*2.0-t6.*t11.*t24.*t198.*4.0-t6.*t11.*t22.*t285.*4.0-dq1.*dq6.*t3.*t4.*t9.*4.0-dq1.*dq5.*t3.*t5.*t23.*2.0-dq1.*dq5.*t3.*t5.*t25.*4.0+dq2.*dq4.*t10.*t23.*t25.*8.0+dq2.*dq6.*t23.*t24.*t25.*4.0;
et61 = t3.*t6.*t8.*t11.*t12.*-2.0-t4.*t6.*t11.*t24.*t45.*4.0+t5.*t6.*t9.*t11.*t209.*4.0+dq2.*dq5.*t5.*t6.*t10.*t11.*4.0+dq1.*dq6.*t3.*t4.*t9.*t24.*2.0+dq1.*dq6.*t3.*t4.*t9.*t25.*8.0-dq1.*dq4.*t5.*t8.*t9.*t25.*4.0+dq1.*dq5.*t3.*t5.*t23.*t25.*4.0-dq2.*dq5.*t5.*t6.*t10.*t11.*t23.*4.0-dq1.*dq6.*t3.*t4.*t9.*t24.*t25.*4.0+dq1.*dq4.*t4.*t5.*t6.*t8.*t10.*t11.*4.0;
et62 = -t11.*t42-t11.*t77-t11.*t100+t11.*t320-dq2.*dq5.*t11.*2.0+ddq6.*t4.*t6-t4.*t11.*t16-t5.*t6.*t32+t6.*t9.*t37-t6.*t9.*t56+t4.*t11.*t58+t6.*t9.*t61.*2.0+t11.*t24.*t42.*2.0+t4.*t6.*t87+t11.*t24.*t77.*2.0+t11.*t24.*t98.*2.0-t9.*t11.*t114.*2.0+t11.*t24.*t100.*2.0-t9.*t11.*t117.*2.0-t4.*t6.*t128.*2.0+t4.*t6.*t161+t9.*t11.*t228.*2.0-t6.*t9.*t256.*2.0-t6.*t9.*t432.*2.0-dq2.*dq4.*t5.*t6.*2.0-dq4.*dq6.*t6.*t9.*2.0+dq2.*dq5.*t11.*t23.*2.0+dq2.*dq5.*t11.*t24.*4.0+ddq2.*t5.*t10.*t11.*2.0+ddq6.*t9.*t10.*t11+t6.*t9.*t10.*t12+t6.*t9.*t10.*t14+t6.*t9.*t10.*t16+t5.*t6.*t23.*t32.*2.0-t5.*t10.*t11.*t47.*4.0-t5.*t10.*t11.*t93.*2.0;
et63 = t5.*t6.*t9.*t113.*-4.0-t9.*t10.*t11.*t120.*4.0-t11.*t22.*t24.*t98.*4.0+t9.*t11.*t24.*t114.*4.0+t5.*t10.*t11.*t198.*4.0+t5.*t6.*t9.*t210.*2.0+t5.*t10.*t11.*t369.*2.0+dq1.*dq5.*t3.*t6.*t10.*2.0-dq1.*dq4.*t4.*t8.*t11.*2.0+dq2.*dq6.*t5.*t6.*t10.*2.0-dq1.*dq6.*t6.*t8.*t9.*2.0+dq4.*dq6.*t4.*t10.*t11.*2.0+dq2.*dq4.*t5.*t6.*t23.*4.0+dq4.*dq6.*t6.*t9.*t24.*2.0-dq2.*dq5.*t11.*t23.*t24.*4.0+t4.*t5.*t10.*t11.*t45.*4.0+t3.*t5.*t8.*t10.*t11.*t12.*2.0+dq1.*dq4.*t6.*t8.*t9.*t10.*2.0+dq1.*dq6.*t4.*t8.*t10.*t11.*2.0-dq1.*dq5.*t3.*t6.*t10.*t23.*2.0-dq1.*dq6.*t3.*t5.*t11.*t23.*2.0+dq1.*dq4.*t4.*t8.*t11.*t24.*4.0-dq2.*dq6.*t5.*t6.*t10.*t23.*2.0+dq1.*dq6.*t6.*t8.*t9.*t24.*2.0;
et64 = -t6.*t42-t6.*t77-t6.*t100+t6.*t320-dq2.*dq5.*t6.*2.0-ddq6.*t4.*t11-t4.*t6.*t16+t5.*t11.*t32+t4.*t11.*t43+t4.*t6.*t58+t6.*t24.*t42.*2.0+t9.*t11.*t56-t9.*t11.*t61.*2.0+t4.*t11.*t78+t9.*t11.*t85+t6.*t24.*t77.*2.0+t6.*t24.*t98.*2.0-t6.*t9.*t114.*2.0+t6.*t24.*t100.*2.0-t6.*t9.*t117.*2.0+t4.*t11.*t128.*2.0+t6.*t9.*t228.*2.0+t9.*t11.*t256.*2.0+t9.*t11.*t432.*2.0+dq2.*dq4.*t5.*t11.*2.0+dq4.*dq6.*t9.*t11.*2.0+dq2.*dq5.*t6.*t23.*2.0+dq2.*dq5.*t6.*t24.*4.0+ddq2.*t5.*t6.*t10.*2.0+ddq6.*t6.*t9.*t10-t9.*t10.*t11.*t14-t9.*t10.*t11.*t16-t5.*t6.*t10.*t47.*4.0-t5.*t11.*t23.*t32.*2.0+t9.*t10.*t11.*t58-t5.*t6.*t10.*t93.*2.0+t5.*t9.*t11.*t113.*4.0;
et65 = t6.*t9.*t10.*t120.*-4.0-t6.*t22.*t24.*t98.*4.0+t6.*t9.*t24.*t114.*4.0+t5.*t6.*t10.*t198.*4.0-t5.*t9.*t11.*t210.*2.0+t5.*t6.*t10.*t369.*2.0-dq1.*dq4.*t4.*t6.*t8.*2.0-dq1.*dq5.*t3.*t10.*t11.*2.0+dq4.*dq6.*t4.*t6.*t10.*2.0-dq2.*dq6.*t5.*t10.*t11.*2.0+dq1.*dq6.*t8.*t9.*t11.*2.0-dq2.*dq4.*t5.*t11.*t23.*4.0-dq4.*dq6.*t9.*t11.*t24.*2.0-dq2.*dq5.*t6.*t23.*t24.*4.0+t4.*t5.*t6.*t10.*t45.*4.0+t3.*t5.*t6.*t8.*t10.*t12.*2.0+dq1.*dq6.*t4.*t6.*t8.*t10.*2.0-dq1.*dq4.*t8.*t9.*t10.*t11.*2.0-dq1.*dq6.*t3.*t5.*t6.*t23.*2.0+dq1.*dq4.*t4.*t6.*t8.*t24.*4.0+dq1.*dq5.*t3.*t10.*t11.*t23.*2.0+dq2.*dq6.*t5.*t10.*t11.*t23.*2.0-dq1.*dq6.*t8.*t9.*t11.*t24.*2.0;
et66 = ddq2-t93-t94-t95+t104+t106+t108+t109-t118+t121+t132+t138+t154+t165-t212+t225+t227+t231+t235+t237+t243+t245-t252+t263+t264+t268+t285+t287-t296-t310+t319+t360+t363+t369+t371-t392-t396-t399-t402-t403-t406-t408+t411+t416-t445+t446+t450+t481-t486-t510+t516+t519+t520+t539+t557+t571+t572+t577-t584+t600+t616+t617+t620+t622+t632+t635+t638-t649+t657+t668+t681-t685+t686-t24.*t198.*2.0+t24.*t269+t25.*t276+t25.*t420+t25.*t423+t25.*t466+t25.*t467+t25.*t490+t24.*t494-t4.*t24.*t45.*2.0-t24.*t25.*t47.*2.0-t24.*t25.*t126.*2.0+t3.*t8.*t24.*t58-t5.*t9.*t25.*t209.*2.0;
et67 = dq2.*dq4.*t6.*t10.*t11.*-2.0+t5.*t6.*t9.*t11.*t58-t6.*t9.*t10.*t11.*t113.*4.0-dq1.*dq5.*t3.*t5.*t6.*t11.*2.0-dq1.*dq4.*t5.*t6.*t8.*t9.*t11.*2.0-dq1.*dq6.*t3.*t4.*t6.*t9.*t11.*t24.*2.0;
et68 = t36+t49+t93+t95+t104-t109+t118-t121+t130-t165+t204+t212+t225-t231-t237-t245+t252+t269+t296+t310+t312-t319+t322+t329-t360-t363+t392+t396+t402+t403+t406+t408-t416+t436+t438+t444+t445-t481+t486+t494+t505+t510-t519+t525+t526+t534-t539+t545+t546-t557-t572-t577-t617+t624+t627-t632+t643+t649-t657+t673+t676-t681+t685+t9.*t11.*t160-t24.*t25.*t198.*2.0+t24.*t25.*t269+t9.*t11.*t313+t24.*t25.*t494+t3.*t8.*t25.*t58-t4.*t24.*t25.*t45.*2.0-t4.*t5.*t6.*t11.*t46.*2.0+t3.*t8.*t24.*t25.*t58-dq2.*dq4.*t6.*t10.*t11.*t23.*4.0-dq2.*dq5.*t5.*t10.*t23.*t25.*2.0-dq2.*dq6.*t6.*t11.*t23.*t24.*2.0;
et69 = dq1.*dq5.*t3.*t5.*t6.*t11.*t23.*-2.0;
et70 = ddq4.*t6.*1.82e-2+t6.*t39.*1.82e-2-t11.*t34.*1.56e-2+t11.*t37.*9.1e-3+t6.*t46.*3.64e-2+t11.*t55.*9.1e-3-t11.*t56.*9.1e-3+t11.*t61.*9.1e-3+t11.*t65.*1.56e-2+t10.*t72.*1.56e-2-t6.*t96.*1.82e-2+t6.*t114.*3.64e-2-t11.*t125.*3.12e-2+t10.*t137.*1.56e-2-t11.*t140.*9.1e-3-t6.*t152.*1.82e-2-t6.*t172.*1.82e-2;
et71 = t6.*t176.*1.82e-2-t6.*t228.*1.82e-2-t11.*t256.*9.1e-3-t11.*t284.*1.56e-2-t6.*t372.*1.82e-2-t6.*t376.*1.82e-2+t11.*t432.*9.1e-3+t10.*t441.*1.56e-2-t6.*t528.*1.82e-2+t6.*t601.*1.82e-2-dq4.*dq6.*t11.*1.82e-2-ddq6.*t6.*t10.*9.1e-3+q3.*t11.*t34-q3.*t10.*t72+q3.*t11.*t125.*2.0-q3.*t10.*t137+q3.*t11.*t157+q3.*t11.*t284+q3.*t10.*t541+t10.*t11.*t16.*9.1e-3;
et72 = t6.*t10.*t51.*3.64e-2-t6.*t24.*t46.*3.64e-2+t6.*t23.*t48.*3.64e-2-t11.*t23.*t55.*1.82e-2+t4.*t11.*t76+t6.*t10.*t120.*3.64e-2+t5.*t11.*t125.*1.82e-2-t6.*t24.*t114.*3.64e-2+t5.*t11.*t129.*1.82e-2+t6.*t10.*t207.*3.64e-2+t5.*t11.*t210.*1.82e-2+t11.*t23.*t256.*1.82e-2+dq2.*dq3.*t4.*t11.*2.0-dq1.*dq6.*t8.*t11.*1.82e-2+dq4.*dq6.*t11.*t24.*1.82e-2-g.*t7.*t9.*t11+q3.*t6.*t10.*t184-t6.*t9.*t10.*t76;
et73 = t6.*t23.*t24.*t48.*(-3.64e-2)+t4.*t9.*t11.*t119.*3.64e-2-dq1.*dq3.*t3.*t9.*t11.*2.0-dq2.*dq3.*t6.*t9.*t10.*2.0-dq2.*dq5.*t4.*t10.*t11.*1.82e-2+dq1.*dq6.*t8.*t11.*t24.*1.82e-2-g.*t4.*t6.*t7.*t10-dq1.*dq3.*t3.*t4.*t6.*t10.*2.0-dq1.*dq2.*t4.*t6.*t8.*t10.*3.12e-2+dq1.*dq5.*t3.*t9.*t10.*t11.*1.82e-2;
et74 = ddq4.*t11.*1.82e-2+t6.*t34.*1.56e-2-t6.*t37.*9.1e-3+t11.*t39.*1.82e-2+t11.*t46.*3.64e-2-t6.*t55.*9.1e-3+t6.*t56.*9.1e-3-t6.*t61.*9.1e-3-t6.*t65.*1.56e-2+t11.*t80.*1.56e-2-t11.*t96.*1.82e-2+t11.*t114.*3.64e-2+t6.*t125.*3.12e-2+t6.*t140.*9.1e-3+t11.*t139.*1.56e-2-t11.*t152.*1.82e-2-t11.*t172.*1.82e-2;
et75 = t11.*t176.*1.82e-2-t11.*t228.*1.82e-2+t6.*t256.*9.1e-3+t6.*t284.*1.56e-2-t11.*t372.*1.82e-2-t11.*t376.*1.82e-2-t6.*t432.*9.1e-3+t11.*t460.*1.56e-2-t11.*t528.*1.82e-2+t11.*t601.*1.82e-2+dq4.*dq6.*t6.*1.82e-2-ddq6.*t10.*t11.*9.1e-3-q3.*t6.*t34+q3.*t6.*t65-q3.*t11.*t80-q3.*t6.*t125.*2.0-q3.*t11.*t139+q3.*t6.*t465-t6.*t10.*t16.*9.1e-3+t10.*t11.*t51.*3.64e-2;
et76 = t11.*t24.*t46.*(-3.64e-2)+t11.*t23.*t48.*3.64e-2+t6.*t23.*t55.*1.82e-2-t4.*t6.*t76-t5.*t6.*t125.*1.82e-2-t5.*t6.*t129.*1.82e-2+t10.*t11.*t120.*3.64e-2-t11.*t24.*t114.*3.64e-2-t5.*t6.*t210.*1.82e-2+t10.*t11.*t207.*3.64e-2-t6.*t23.*t256.*1.82e-2-dq2.*dq3.*t4.*t6.*2.0+dq1.*dq6.*t6.*t8.*1.82e-2-dq4.*dq6.*t6.*t24.*1.82e-2+g.*t6.*t7.*t9+q3.*t10.*t11.*t184+q3.*t10.*t11.*t468-t9.*t10.*t11.*t76;
et77 = t11.*t23.*t24.*t48.*(-3.64e-2)-t4.*t6.*t9.*t119.*3.64e-2+dq1.*dq3.*t3.*t6.*t9.*2.0+dq2.*dq5.*t4.*t6.*t10.*1.82e-2-dq2.*dq3.*t9.*t10.*t11.*2.0-dq1.*dq6.*t6.*t8.*t24.*1.82e-2-g.*t4.*t7.*t10.*t11-dq1.*dq3.*t3.*t4.*t10.*t11.*2.0-dq1.*dq5.*t3.*t6.*t9.*t10.*1.82e-2-dq1.*dq2.*t4.*t8.*t10.*t11.*3.12e-2;
et78 = -t55+t56+t85+t140+t155+t189+t256-t303+t326+t346-t448-t581+t25.*t37.*2.0+t25.*t55.*2.0-t25.*t56.*2.0+t25.*t61.*2.0-t5.*t129.*2.0-t25.*t140.*2.0-t5.*t210.*2.0-t25.*t256.*2.0+t25.*t432.*2.0+t5.*t465-dq4.*dq6.*t24.*2.0-t6.*t11.*t46.*4.0+t6.*t11.*t48.*4.0-t6.*t11.*t53.*4.0-t23.*t25.*t55.*4.0+t6.*t11.*t96.*2.0-t6.*t11.*t114.*4.0-t6.*t11.*t117.*4.0+t5.*t25.*t125.*4.0+t5.*t25.*t129.*4.0+t6.*t11.*t152.*2.0+t6.*t11.*t172.*2.0-t6.*t11.*t176.*4.0+t6.*t11.*t211.*4.0+t5.*t25.*t210.*4.0+t6.*t11.*t228.*2.0+t23.*t25.*t256.*4.0+t6.*t11.*t372.*4.0+t6.*t11.*t376.*2.0+t6.*t11.*t528.*2.0-t6.*t11.*t601.*2.0-dq1.*dq6.*t8.*t24.*2.0+dq4.*dq6.*t24.*t25.*4.0;
et79 = t6.*t10.*t11.*t51.*-4.0+t6.*t11.*t24.*t46.*4.0-t6.*t11.*t23.*t48.*8.0-t6.*t10.*t11.*t120.*4.0+t6.*t11.*t24.*t114.*4.0+t4.*t9.*t25.*t119.*8.0-t6.*t10.*t11.*t207.*4.0-dq2.*dq5.*t4.*t10.*t25.*4.0+dq1.*dq6.*t8.*t24.*t25.*4.0+t6.*t11.*t23.*t24.*t48.*4.0+dq1.*dq5.*t3.*t9.*t10.*t25.*4.0;
et80 = ddq5.*t6.*1.82e-2+t6.*t34.*1.82e-2+t11.*t35.*9.1e-3-t6.*t45.*3.64e-2+t6.*t52.*1.82e-2-t6.*t55.*1.56e-2-t6.*t61.*1.56e-2-t6.*t65.*1.82e-2+t11.*t67.*9.1e-3+t11.*t80.*9.1e-3-t6.*t113.*3.64e-2+t6.*t122.*1.82e-2+t6.*t129.*1.82e-2+t6.*t140.*1.56e-2+t11.*t139.*9.1e-3+t6.*t210.*1.82e-2-t6.*t256.*1.56e-2;
et81 = t6.*t284.*(-1.82e-2)+t10.*t349.*1.82e-2-t6.*t377.*1.82e-2-t6.*t432.*1.56e-2-t11.*t460.*9.1e-3+t11.*t544.*9.1e-3-dq5.*dq6.*t11.*1.82e-2-ddq3.*t6.*t10+q3.*t6.*t55+q3.*t6.*t61-q3.*t6.*t140+q3.*t6.*t256+q3.*t6.*t303+q3.*t6.*t432+t5.*t11.*t48.*1.82e-2+t5.*t6.*t55.*1.82e-2+t6.*t24.*t45.*3.64e-2+t6.*t10.*t64-t5.*t6.*t125.*3.12e-2+t6.*t24.*t113.*3.64e-2+t6.*t24.*t125.*3.64e-2;
et82 = t4.*t9.*t178.*(-9.1e-3)+t6.*t24.*t284.*3.64e-2+t10.*t23.*t349.*1.82e-2-dq2.*dq6.*t4.*t11.*1.82e-2-t5.*t6.*t10.*t12.*1.82e-2-t5.*t6.*t10.*t14.*1.82e-2-t9.*t10.*t11.*t49.*1.82e-2-t5.*t11.*t23.*t48.*1.82e-2+t4.*t5.*t6.*t76+dq2.*dq3.*t4.*t5.*t6.*2.0+dq1.*dq6.*t3.*t9.*t11.*1.82e-2+dq2.*dq4.*t4.*t10.*t11.*1.82e-2-g.*t5.*t6.*t7.*t9+t4.*t5.*t6.*t9.*t119.*3.64e-2-dq1.*dq3.*t3.*t5.*t6.*t9.*2.0-dq1.*dq4.*t5.*t6.*t8.*t10.*3.64e-2;
et83 = ddq5.*t11.*1.82e-2-t6.*t35.*9.1e-3+t11.*t34.*1.82e-2-t11.*t45.*3.64e-2+t11.*t52.*1.82e-2-t11.*t55.*1.56e-2-t11.*t61.*1.56e-2-t6.*t67.*9.1e-3-t11.*t65.*1.82e-2-t10.*t72.*9.1e-3-t11.*t113.*3.64e-2+t11.*t122.*1.82e-2+t11.*t129.*1.82e-2-t10.*t137.*9.1e-3+t11.*t140.*1.56e-2+t11.*t210.*1.82e-2-t11.*t256.*1.56e-2;
et84 = t11.*t284.*(-1.82e-2)+t11.*t373.*1.82e-2-t11.*t377.*1.82e-2-t11.*t432.*1.56e-2+t10.*t441.*9.1e-3-t6.*t544.*9.1e-3+t11.*t602.*1.82e-2+dq5.*dq6.*t6.*1.82e-2-ddq3.*t10.*t11+q3.*t11.*t55+q3.*t11.*t61-q3.*t11.*t140+q3.*t11.*t256+q3.*t11.*t303+q3.*t11.*t432-t5.*t6.*t48.*1.82e-2+t5.*t11.*t55.*1.82e-2+t11.*t24.*t45.*3.64e-2+t10.*t11.*t64-t5.*t11.*t125.*3.12e-2+t11.*t24.*t113.*3.64e-2;
et85 = t11.*t24.*t125.*3.64e-2+t4.*t9.*t166.*9.1e-3+t11.*t24.*t284.*3.64e-2+dq2.*dq6.*t4.*t6.*1.82e-2-t5.*t10.*t11.*t12.*1.82e-2-t5.*t10.*t11.*t14.*1.82e-2+t6.*t9.*t10.*t49.*1.82e-2+t5.*t6.*t23.*t48.*1.82e-2+t4.*t5.*t11.*t76-dq1.*dq6.*t3.*t6.*t9.*1.82e-2+dq2.*dq3.*t4.*t5.*t11.*2.0-dq2.*dq4.*t4.*t6.*t10.*1.82e-2-g.*t5.*t7.*t9.*t11+t4.*t5.*t9.*t11.*t119.*3.64e-2-dq1.*dq3.*t3.*t5.*t9.*t11.*2.0-dq1.*dq4.*t5.*t8.*t10.*t11.*3.64e-2;
et86 = -t35-t67-t80-t139-t169+t286+t304+t350+t460+dq5.*dq6.*2.0-ddq5.*t29+t25.*t35.*2.0+t25.*t67.*2.0+t25.*t80.*2.0+t25.*t139.*2.0-t5.*t300.*2.0-t25.*t286.*2.0-t25.*t460.*2.0+t5.*t590+t5.*t650+dq2.*dq6.*t4.*2.0-dq5.*dq6.*t25.*4.0-t6.*t11.*t34.*2.0+t6.*t11.*t45.*4.0-t6.*t11.*t52.*4.0+t5.*t25.*t48.*4.0+t6.*t11.*t65.*2.0+t6.*t11.*t113.*4.0-t6.*t11.*t122.*4.0-t6.*t11.*t129.*4.0-t6.*t11.*t210.*4.0+t6.*t11.*t284.*2.0-t10.*t11.*t349.*2.0+t4.*t9.*t421-dq1.*dq6.*t3.*t9.*2.0-dq2.*dq4.*t4.*t10.*2.0-dq2.*dq6.*t4.*t25.*4.0-t6.*t11.*t24.*t45.*4.0-t9.*t10.*t25.*t49.*4.0-t5.*t23.*t25.*t48.*4.0-t6.*t11.*t24.*t113.*4.0;
et87 = t6.*t11.*t24.*t125.*-4.0-t6.*t11.*t24.*t284.*4.0-t10.*t11.*t23.*t349.*2.0+dq1.*dq6.*t3.*t9.*t25.*4.0+dq2.*dq4.*t4.*t10.*t25.*4.0+t5.*t6.*t10.*t11.*t12.*2.0+t5.*t6.*t10.*t11.*t14.*2.0-t4.*t5.*t6.*t9.*t11.*t119.*4.0+dq1.*dq4.*t5.*t6.*t8.*t10.*t11.*4.0;
et88 = t72.*(-1.56e-2)-t137.*1.56e-2+t153.*1.56e-2-t178.*1.56e-2-t265.*1.56e-2-t374.*1.56e-2-t441.*1.56e-2+t529.*1.56e-2+q3.*t72+q3.*t137-q3.*t153+q3.*t178+q3.*t265+q3.*t374+q3.*t441+t11.*t12.*9.1e-3+t11.*t14.*9.1e-3+t11.*t15.*9.1e-3-t6.*t43.*9.1e-3-t6.*t51.*1.82e-2+t6.*t70.*9.1e-3-t6.*t78.*9.1e-3-t6.*t120.*1.82e-2;
et89 = t6.*t128.*(-1.82e-2)+t6.*t136.*9.1e-3-t6.*t207.*1.82e-2-t6.*t209.*1.82e-2-t6.*t299.*9.1e-3+t6.*t440.*9.1e-3+t6.*t561.*9.1e-3-ddq3.*t5.*t11-t11.*t12.*t24.*9.1e-3+t11.*t13.*t23.*9.1e-3+t11.*t13.*t24.*9.1e-3-t11.*t14.*t24.*9.1e-3+t5.*t11.*t64+t6.*t9.*t76+t10.*t11.*t125.*3.12e-2-t6.*t23.*t119.*1.82e-2-t11.*t23.*t150.*9.1e-3;
et90 = t11.*t24.*t150.*9.1e-3-t10.*t11.*t432.*1.82e-2+dq2.*dq3.*t6.*t9.*2.0+dq2.*dq5.*t4.*t11.*1.82e-2+dq1.*dq4.*t8.*t11.*1.82e-2+g.*t4.*t6.*t7-q3.*t10.*t11.*t125.*2.0+q3.*t10.*t11.*t465-t5.*t10.*t11.*t45.*1.82e-2-t11.*t13.*t23.*t24.*9.1e-3-t4.*t9.*t11.*t48.*1.82e-2-t4.*t10.*t11.*t76-t5.*t10.*t11.*t113.*1.82e-2-t5.*t10.*t11.*t125.*1.82e-2+t11.*t23.*t24.*t150.*9.1e-3+dq1.*dq3.*t3.*t4.*t6.*2.0+dq1.*dq2.*t4.*t6.*t8.*3.12e-2;
et91 = dq1.*dq5.*t3.*t9.*t11.*(-1.82e-2)-dq2.*dq3.*t4.*t10.*t11.*2.0-dq1.*dq4.*t8.*t11.*t24.*1.82e-2+g.*t7.*t9.*t10.*t11+t4.*t9.*t11.*t24.*t48.*1.82e-2-dq1.*dq2.*q3.*t4.*t6.*t8.*2.0+dq1.*dq3.*t3.*t9.*t10.*t11.*2.0;
et92 = t81.*(-1.56e-2)-t143.*1.56e-2-t147.*1.56e-2+t166.*1.56e-2+t251.*1.56e-2+t349.*1.56e-2-t461.*1.56e-2-t513.*1.56e-2+q3.*t81+q3.*t143+q3.*t147-q3.*t166-q3.*t251+q3.*t461+q3.*t492+q3.*t513-t6.*t12.*9.1e-3-t6.*t14.*9.1e-3-t6.*t15.*9.1e-3-t11.*t43.*9.1e-3-t11.*t51.*1.82e-2+t11.*t70.*9.1e-3-t11.*t78.*9.1e-3;
et93 = t11.*t120.*(-1.82e-2)-t11.*t128.*1.82e-2+t11.*t136.*9.1e-3-t11.*t207.*1.82e-2-t11.*t209.*1.82e-2-t11.*t299.*9.1e-3+t11.*t440.*9.1e-3+t11.*t561.*9.1e-3+ddq3.*t5.*t6+t6.*t12.*t24.*9.1e-3-t6.*t13.*t23.*9.1e-3-t6.*t13.*t24.*9.1e-3+t6.*t14.*t24.*9.1e-3-t5.*t6.*t64+t9.*t11.*t76-t6.*t10.*t125.*3.12e-2-t11.*t23.*t119.*1.82e-2;
et94 = t6.*t23.*t150.*9.1e-3-t6.*t24.*t150.*9.1e-3+t6.*t10.*t432.*1.82e-2-dq2.*dq5.*t4.*t6.*1.82e-2-dq1.*dq4.*t6.*t8.*1.82e-2+dq2.*dq3.*t9.*t11.*2.0+g.*t4.*t7.*t11+q3.*t6.*t10.*t125.*2.0+t5.*t6.*t10.*t45.*1.82e-2+t6.*t13.*t23.*t24.*9.1e-3+t4.*t6.*t9.*t48.*1.82e-2+t4.*t6.*t10.*t76+t5.*t6.*t10.*t113.*1.82e-2+t5.*t6.*t10.*t125.*1.82e-2-t6.*t23.*t24.*t150.*9.1e-3+dq1.*dq3.*t3.*t4.*t11.*2.0+dq1.*dq5.*t3.*t6.*t9.*1.82e-2+dq2.*dq3.*t4.*t6.*t10.*2.0;
et95 = dq1.*dq2.*t4.*t8.*t11.*3.12e-2+dq1.*dq4.*t6.*t8.*t24.*1.82e-2-g.*t6.*t7.*t9.*t10-t4.*t6.*t9.*t24.*t48.*1.82e-2-dq1.*dq2.*q3.*t4.*t8.*t11.*2.0-dq1.*dq3.*t3.*t6.*t9.*t10.*2.0;
et96 = t13-t15+t273+t274+t289+t488+t12.*t24-t13.*t24-t13.*t25.*2.0+t14.*t24+t15.*t25.*2.0+t25.*t150.*2.0+t24.*t273+t10.*t303+t10.*t432.*2.0-dq2.*dq5.*t4.*2.0+t5.*t10.*t45.*2.0+t13.*t23.*t24-t12.*t24.*t25.*2.0+t13.*t23.*t25.*4.0+t13.*t24.*t25.*2.0-t14.*t24.*t25.*2.0+t6.*t11.*t51.*4.0+t5.*t10.*t113.*2.0+t6.*t11.*t115.*4.0-t6.*t11.*t119.*4.0+t6.*t11.*t120.*4.0+t6.*t11.*t128.*4.0-t23.*t25.*t150.*4.0+t24.*t25.*t150.*2.0+t6.*t11.*t207.*4.0-t6.*t11.*t208.*4.0+t6.*t11.*t209.*4.0+t6.*t11.*t299.*4.0+t23.*t24.*t273+t24.*t25.*t289-t6.*t11.*t440.*4.0-t10.*t25.*t432.*4.0+t24.*t25.*t488-t6.*t11.*t561.*4.0+dq1.*dq5.*t3.*t9.*2.0+dq2.*dq5.*t4.*t25.*4.0+dq1.*dq4.*t8.*t24.*2.0-t4.*t9.*t24.*t48.*2.0;
et97 = t5.*t10.*t25.*t45.*-4.0-t13.*t23.*t24.*t25.*2.0-t4.*t9.*t25.*t48.*8.0-t5.*t10.*t25.*t113.*4.0+t6.*t11.*t23.*t119.*8.0-t5.*t10.*t25.*t125.*4.0-dq1.*dq5.*t3.*t9.*t25.*4.0-dq1.*dq4.*t8.*t24.*t25.*4.0;
mt1 = [et1+et2+et3+et4+et5+et6+et7+et8+et9+et10,et41+et42+et43+et44+et45+et46+et47,-t75+t160+t162-t166-t168+t251+t271+t272+t313+t336+t435+t461+t492+t513+t6.*t10.*t45.*2.0+t9.*t11.*t49.*2.0+t6.*t10.*t113.*2.0-t9.*t11.*t121.*2.0-dq2.*dq4.*t4.*t11.*2.0-dq2.*dq6.*t6.*t9.*2.0+dq5.*dq6.*t10.*t11.*2.0-dq1.*dq6.*t3.*t4.*t6.*2.0+dq2.*dq6.*t4.*t10.*t11.*2.0,et70+et71+et72+et73,et80+et81+et82,et88+et89+et90+et91,et11+et12+et13+et14+et15+et16+et17+et18+et19+et20,et48+et49+et50+et51+et52+et53+et54];
mt2 = [t63+t72-t83+t137-t153-t181+t265+t316+t317+t452+t529+t541+t11.*t421-t6.*t9.*t49.*2.0+t10.*t11.*t45.*2.0+t10.*t11.*t113.*2.0+t6.*t9.*t121.*2.0+dq2.*dq4.*t4.*t6.*2.0-dq5.*dq6.*t6.*t10.*2.0-dq2.*dq6.*t9.*t11.*2.0-dq1.*dq6.*t3.*t4.*t11.*2.0-dq2.*dq5.*t4.*t5.*t11.*2.0-dq2.*dq6.*t4.*t6.*t10.*2.0,et74+et75+et76+et77,et83+et84+et85,et92+et93+et94+et95,(t3.*t422.*(t32.*-2.159e+3+g.*t7.*5.0e+3+t32.*t90+dq1.*dq3.*t3.*1.0e+4+dq1.*dq2.*t8.*4.318e+3-dq1.*dq2.*q3.*t8.*1.0e+4))./2.5e+7];
mt3 = [(q3./5.0e+3-8.636e-5).*(ddq2.*-2.159e+3+t76.*5.0e+3+dq2.*dq3.*1.0e+4+ddq2.*t90-t12.*t26.*1.0795e+3+q3.*t12.*t26.*2.5e+3),ddq3+t13.*4.318e-1-t64+t150.*4.318e-1-q3.*t13+q3.*t273,0.0,0.0,0.0,et21+et22,et55+et56,t55+t56+t85+t140+t155+t189+t256+t346+t432+t5.*t45.*2.0+t5.*t113.*2.0,t5.*t694.*(-4.0e-4)];
mt4 = [t69.*1.56e-2-t99.*1.56e-2-t151.*1.56e-2-t239.*1.56e-2+t439.*1.56e-2-ddq3.*t5+q3.*t99+q3.*t151+q3.*t158+q3.*t239+t5.*t64+t10.*t125.*3.12e-2-q3.*t10.*t125.*2.0+q3.*t10.*t465-t4.*t10.*t76-dq2.*dq3.*t4.*t10.*2.0+g.*t7.*t9.*t10+dq1.*dq3.*t3.*t9.*t10.*2.0,0.0,et23+et24,et57+et58,t88-t99+t151+t158+t195+t218+t291+t421+t439+t10.*t45.*2.0+t10.*t113.*2.0,t10.*t694.*(-4.0e-4)];
mt5 = [t55.*(-1.56e-2)-t61.*1.56e-2+t140.*1.56e-2-t256.*1.56e-2-t432.*1.56e-2-ddq3.*t10+q3.*t55+q3.*t61-q3.*t140+q3.*t256+q3.*t303+q3.*t432+t10.*t64-t5.*t125.*3.12e-2+t4.*t5.*t76+dq2.*dq3.*t4.*t5.*2.0-g.*t5.*t7.*t9-dq1.*dq3.*t3.*t5.*t9.*2.0,0.0,et25+et26+et27+et28,et59+et60+et61,0.0,et78+et79,et86+et87,et96+et97];
mt6 = [t8.*t34.*1.56e-2-t3.*t42.*1.56e-2-t8.*t65.*3.12e-2+t4.*t86+t9.*t84-t3.*t100.*1.56e-2-t8.*t113.*3.12e-2+dq1.*dq2.*t9.*3.12e-2+ddq3.*t3.*t4-q3.*t8.*t34+q3.*t3.*t42+q3.*t8.*t65.*2.0+q3.*t3.*t100+q3.*t8.*t113.*2.0+t3.*t4.*t13.*1.56e-2-dq1.*dq2.*q3.*t9.*2.0-dq2.*dq3.*t4.*t8.*2.0-dq1.*dq2.*t9.*t22.*(3.9e+1./6.25e+2)-q3.*t3.*t4.*t13+dq1.*dq2.*q3.*t9.*t22.*4.0+dq1.*dq3.*t3.*t8.*t9.*2.0];
mt7 = [ddq4.*t4.*1.56e-2+ddq3.*t9-t9.*t12.*1.56e-2-t9.*t14.*1.56e-2+t4.*t39.*1.56e-2-t9.*t64+t9.*t150.*3.12e-2-ddq4.*q3.*t4+q3.*t9.*t12+q3.*t9.*t14-q3.*t4.*t39-q3.*t9.*t150.*2.0-dq1.*dq4.*t8.*t9.*3.12e-2+dq1.*dq4.*q3.*t8.*t9.*2.0,t40+t59+t468-t9.*t49.*2.0+dq2.*dq4.*t4.*2.0,t34.*1.56e-2-t65.*1.56e-2+t125.*3.12e-2+t284.*1.56e-2-q3.*t34+q3.*t65-q3.*t125.*2.0+q3.*t465-t4.*t76-dq2.*dq3.*t4.*2.0+g.*t7.*t9+dq1.*dq3.*t3.*t9.*2.0,0.0,0.0];
mt8 = [et29+et30+et31,et62+et63,0.0,t75+t160+t162+t166+t168+t251+t271+t272+t313+t336+t435+t492+t24.*t81.*2.0+t24.*t143.*2.0-t23.*t166.*2.0+t11.*t184+t23.*t349.*2.0+t11.*t468+t24.*t461.*2.0+dq4.*dq5.*t11.*2.0-t10.*t11.*t35.*2.0-t6.*t10.*t52.*2.0-t10.*t11.*t67.*2.0-t6.*t10.*t122.*2.0-t6.*t10.*t125.*2.0-t5.*t11.*t128.*4.0-t5.*t11.*t209.*4.0+t5.*t6.*t289-t5.*t11.*t299.*2.0+t6.*t10.*t465+t9.*t11.*t584+dq1.*dq5.*t8.*t11.*2.0-dq4.*dq5.*t11.*t24.*4.0-t5.*t11.*t23.*t119.*4.0+dq2.*dq6.*t6.*t9.*t24.*2.0-dq1.*dq5.*t8.*t11.*t24.*4.0+dq1.*dq6.*t3.*t4.*t6.*t24.*2.0-dq1.*dq2.*t4.*t8.*t11.*t24.*4.0];
mt9 = [ddq6.*t6+t11.*t13-t11.*t14-t11.*t16+t11.*t58+t6.*t70+t6.*t87+t6.*t115.*2.0-t6.*t119.*2.0+t6.*t136+t11.*t150+t6.*t161-t6.*t208.*2.0+t6.*t299+t6.*t387+t6.*t540+t6.*t646+t11.*t12.*t24.*2.0-t11.*t13.*t23-t11.*t13.*t24.*2.0+t11.*t14.*t24.*2.0+t11.*t23.*t150-t11.*t24.*t150.*2.0+t11.*t24.*t201+t10.*t11.*t432.*4.0-dq1.*dq4.*t8.*t11.*2.0+dq4.*dq6.*t10.*t11.*2.0+t5.*t10.*t11.*t45.*4.0+t4.*t9.*t11.*t48.*2.0+t5.*t10.*t11.*t113.*4.0+t5.*t10.*t11.*t125.*4.0-t11.*t23.*t24.*t150.*2.0-dq2.*dq6.*t5.*t9.*t11.*2.0+dq1.*dq6.*t8.*t10.*t11.*2.0+dq1.*dq4.*t8.*t11.*t24.*4.0-t4.*t9.*t11.*t24.*t48.*4.0-dq1.*dq6.*t3.*t4.*t5.*t11.*2.0];
mt10 = [ddq5.*t6+t6.*t34+t11.*t35+t11.*t67+t11.*t80+t6.*t125.*2.0+t11.*t139+t6.*t157+t6.*t284+t6.*t306+t11.*t350+t6.*t377+t11.*t460+t10.*t492+t5.*t11.*t46.*2.0-t5.*t6.*t55-t6.*t24.*t45.*2.0+t5.*t11.*t114.*2.0-t6.*t24.*t113.*2.0-t6.*t24.*t125.*2.0+t4.*t9.*t178-t6.*t24.*t284.*2.0+t10.*t23.*t492-dq4.*dq5.*t10.*t11.*2.0+t5.*t6.*t10.*t12+t5.*t6.*t10.*t14+t4.*t9.*t11.*t421-dq1.*dq5.*t8.*t10.*t11.*2.0-t4.*t5.*t6.*t9.*t119.*2.0-dq1.*dq2.*t4.*t8.*t10.*t11.*2.0];
mt11 = [t60.*1.56e-2+t79.*1.56e-2+t174.*1.56e-2-t177.*1.56e-2-q3.*t60-q3.*t79+q3.*t102-q3.*t174+q3.*t177+q3.*t302+t8.*t59.*3.12e-2+t9.*t86+t4.*t163-dq1.*dq2.*t4.*3.12e-2+ddq3.*t3.*t9-q3.*t8.*t59.*2.0-t8.*t9.*t49.*3.12e-2-dq2.*dq3.*t8.*t9.*2.0+dq1.*dq2.*t4.*t22.*(3.9e+1./6.25e+2)-dq1.*dq2.*q3.*t4.*t22.*4.0-dq1.*dq3.*t3.*t4.*t8.*2.0];
mt12 = [t42.*1.56e-2+t77.*1.56e-2+t98.*1.56e-2+t100.*1.56e-2-ddq3.*t4-q3.*t42-q3.*t77-q3.*t100+q3.*t320+t4.*t64-t22.*t98.*3.12e-2+q3.*t4.*t58+dq1.*dq4.*t4.*t8.*3.12e-2-dq1.*dq4.*q3.*t4.*t8.*2.0,-t34+t45.*2.0+t65+t113.*2.0+t284,t40.*1.56e-2+t59.*1.56e-2+t297.*1.56e-2-q3.*t40-q3.*t59+q3.*t184+q3.*t468-t9.*t76-dq2.*dq3.*t9.*2.0-g.*t4.*t7-dq1.*dq3.*t3.*t4.*2.0-dq1.*dq2.*t4.*t8.*3.12e-2,0.0,0.0,et32+et33+et34];
mt13 = [et64+et65,0.0,t63-t72+t83-t137+t153+t181-t265+t293+t316+t317+t374+t529+t541+t24.*t72.*2.0+t24.*t137.*2.0+t6.*t184+t23.*t178.*2.0-t23.*t374.*2.0+t24.*t441.*2.0+dq4.*dq5.*t6.*2.0-t6.*t10.*t35.*2.0+t10.*t11.*t52.*2.0-t6.*t10.*t67.*2.0-t5.*t6.*t128.*4.0+t10.*t11.*t122.*2.0+t10.*t11.*t125.*2.0-t5.*t6.*t209.*4.0-t5.*t6.*t299.*2.0+t6.*t9.*t584+dq1.*dq5.*t6.*t8.*2.0-dq4.*dq5.*t6.*t24.*4.0-t5.*t6.*t23.*t119.*4.0-dq1.*dq5.*t6.*t8.*t24.*4.0-dq2.*dq6.*t9.*t11.*t24.*2.0-t4.*t5.*t9.*t11.*t48.*4.0-dq1.*dq5.*t3.*t5.*t9.*t11.*2.0-dq1.*dq2.*t4.*t6.*t8.*t24.*4.0-dq1.*dq6.*t3.*t4.*t11.*t24.*2.0];
mt14 = [-ddq6.*t11+t6.*t13-t6.*t14-t6.*t16+t11.*t43+t6.*t58-t11.*t70+t11.*t78-t11.*t115.*2.0+t11.*t119.*2.0-t11.*t136+t6.*t150+t11.*t208.*2.0-t11.*t299+t11.*t440+t11.*t561+t6.*t12.*t24.*2.0-t6.*t13.*t23-t6.*t13.*t24.*2.0+t6.*t14.*t24.*2.0-t11.*t23.*t119.*2.0+t6.*t23.*t150-t6.*t24.*t150.*2.0+t6.*t24.*t201+t6.*t10.*t432.*4.0-dq1.*dq4.*t6.*t8.*2.0+dq4.*dq6.*t6.*t10.*2.0+t5.*t6.*t10.*t45.*4.0+t4.*t6.*t9.*t48.*2.0+t5.*t6.*t10.*t113.*4.0+t5.*t6.*t10.*t125.*4.0-t6.*t23.*t24.*t150.*2.0-dq2.*dq6.*t5.*t6.*t9.*2.0+dq1.*dq6.*t6.*t8.*t10.*2.0+dq1.*dq4.*t6.*t8.*t24.*4.0-t4.*t6.*t9.*t24.*t48.*4.0-dq1.*dq6.*t3.*t4.*t5.*t6.*2.0];
mt15 = [-ddq5.*t11+t6.*t35-t11.*t34+t6.*t67+t11.*t65+t10.*t72-t11.*t125.*2.0+t10.*t137+t11.*t258+t6.*t350+t11.*t351+t11.*t373+t11.*t410+t10.*t441+t11.*t465+t11.*t497+t11.*t515+t11.*t583+t11.*t602+t5.*t6.*t46.*2.0+t5.*t11.*t55+t5.*t6.*t114.*2.0+t4.*t9.*t166+t4.*t9.*t492-dq4.*dq5.*t6.*t10.*2.0-t5.*t10.*t11.*t14+t5.*t10.*t11.*t58-dq1.*dq5.*t6.*t8.*t10.*2.0-dq1.*dq2.*t4.*t6.*t8.*t10.*2.0-dq1.*dq4.*t5.*t8.*t10.*t11.*2.0,(t3.*(t32.*-3.9e+1+g.*t7.*1.25e+3+q3.*t32.*2.5e+3+dq1.*dq3.*t3.*2.5e+3+dq1.*dq2.*t8.*7.8e+1-dq1.*dq2.*q3.*t8.*5.0e+3))./1.25e+3];
mt16 = [ddq2.*(-3.12e-2)+t76+dq2.*dq3.*2.0+ddq2.*q3.*2.0-t12.*t26.*1.56e-2+q3.*t12.*t26,-t13+t58+t12.*t30,0.0,0.0,0.0,t163+ddq1.*t26.*4.318e-1+dq1.*dq2.*t21.*8.636e-1-dq1.*dq3.*t26-ddq1.*q3.*t26-dq1.*dq2.*q3.*t21.*2.0,-ddq3+t12.*4.318e-1+t64-t150.*8.636e-1+q3.*t58+q3.*t150.*2.0,-ddq2+t329,0.0,0.0,0.0,et35+et36];
mt17 = [-t42-t77-t100-t185+t320-dq2.*dq5.*2.0+ddq2.*t28+t4.*t58+t24.*t42.*2.0+t24.*t77.*2.0+t24.*t98.*2.0-t9.*t114.*2.0+t24.*t100.*2.0+t9.*t228.*2.0+dq2.*dq5.*t23.*2.0+dq2.*dq5.*t24.*4.0-t5.*t10.*t47.*4.0-t5.*t10.*t93.*2.0-t9.*t10.*t120.*4.0-t22.*t24.*t98.*4.0+t9.*t24.*t114.*4.0+t5.*t10.*t198.*4.0+t5.*t10.*t369.*2.0-dq2.*dq5.*t23.*t24.*4.0+t4.*t5.*t10.*t45.*4.0+dq1.*dq4.*t4.*t8.*t24.*4.0+t3.*t5.*t8.*t10.*t12.*2.0,0.0];
mt18 = [-t40-t59+t184+t468+dq4.*dq5.*2.0-ddq4.*t28+t24.*t40.*2.0-t10.*t67.*2.0+t24.*t59.*2.0-t5.*t128.*4.0-t5.*t209.*4.0-t5.*t299.*2.0+t24.*t297.*2.0+t9.*t584+dq1.*dq5.*t8.*2.0-dq4.*dq5.*t24.*4.0-t5.*t23.*t119.*4.0-dq1.*dq5.*t8.*t24.*4.0-dq1.*dq2.*t4.*t8.*t24.*4.0,t13-t14+t58+t150+t12.*t24.*2.0-t13.*t23-t13.*t24.*2.0+t14.*t24.*2.0+t23.*t150-t24.*t150.*2.0+t24.*t201+t10.*t432.*4.0-dq1.*dq4.*t8.*2.0+t5.*t10.*t45.*4.0+t4.*t9.*t48.*2.0+t5.*t10.*t113.*4.0+t5.*t10.*t125.*4.0-t23.*t24.*t150.*2.0+dq1.*dq4.*t8.*t24.*4.0-t4.*t9.*t24.*t48.*4.0,0.0];
mt19 = [-t5.*t33+t5.*t54+t8.*t88+t8.*t151.*2.0+t8.*t158+t8.*t195+t3.*t5.*t36+t3.*t10.*t42+t5.*t23.*t33.*2.0-t3.*t4.*t55-t3.*t4.*t56-t5.*t23.*t54.*2.0+t3.*t10.*t100+t8.*t10.*t113.*2.0+t3.*t9.*t120.*2.0+t5.*t8.*t289-dq1.*dq2.*t9.*t10.*2.0+dq1.*dq4.*t5.*t22.*2.0-t3.*t4.*t5.*t45.*4.0-t4.*t5.*t9.*t91.*2.0-dq2.*dq5.*t4.*t5.*t8.*2.0-dq2.*dq5.*t3.*t10.*t23.*2.0+dq1.*dq2.*t9.*t10.*t22.*4.0-dq1.*dq4.*t5.*t22.*t23.*4.0+dq1.*dq5.*t4.*t9.*t10.*t22.*2.0];
mt20 = [-t5.*t32+t9.*t37-t9.*t56+t9.*t61.*2.0+t4.*t87-t4.*t128.*2.0+t4.*t161-t9.*t256.*2.0-t9.*t432.*2.0-dq2.*dq4.*t5.*2.0+t9.*t10.*t12+t9.*t10.*t14+t5.*t23.*t32.*2.0-t5.*t9.*t113.*4.0+dq1.*dq5.*t3.*t10.*2.0+dq2.*dq4.*t5.*t23.*4.0+dq1.*dq4.*t8.*t9.*t10.*2.0-dq1.*dq5.*t3.*t10.*t23.*2.0,0.0,t88+t99+t151+t158+t195+t218+t291+t421-t23.*t99.*2.0-t10.*t125.*2.0+t23.*t239.*2.0+t5.*t289+t10.*t465,t70+t87+t115.*2.0-t119.*2.0+t136+t161-t208.*2.0+t299+t387+t540+t646,0.0];
mt21 = [-t68+t73+t144-t145+t146+t186+t190-t191+t257+t278-t279+t280-t325+t338+t356-t390-t433-t453+t464-t482-t489-t522+t530-t551-dq2.*dq5.*t4.*t8.*t10.*2.0,-t57+t62-t66+t82+t141-t170-t179+t180+t202+t261+t292-t305+t337+t354-t451+t474-t582+t5.*t9.*t58,0.0,t37+t55-t56+t61-t140-t189+t303+t307-t326+t432+t448+t581+t10.*t273,t35+t67+t80+t139+t169+t188-t286-t304+t544+t10.*t468-t5.*t23.*t48.*2.0,0.0,et37+et38,et66+et67,0.0];
mt22 = [-t46+t48+t96-t110-t114+t135+t149+t152+t172+t211+t219+t228+t230-t241+t250+t260+t262+t300-t301-t308+t321-t331+t353+t355+t359-t362+t372+t376+t407+t409+t475+t506+t508+t528+t532+t535+t538-t556+t568+t569-t590+t594+t597+t623+t642+t684+t687-t10.*t207.*2.0+t25.*t194+t25.*t275+t25.*t314-t25.*t372.*2.0+t25.*t417+t24.*t495+t25.*t496+t25.*t576+t25.*t634-t24.*t25.*t46.*2.0-t24.*t25.*t114.*2.0+t6.*t10.*t11.*t273-dq2.*dq5.*t4.*t6.*t10.*t11.*2.0];
mt23 = [t45-t52+t97-t111+t113-t122+t125-t129+t148+t164-t210+t249+t253-t258-t259+t267+t284-t295+t306+t330-t332+t334-t351-t352+t361+t377+t380-t382+t397-t410+t415+t434+t456+t457-t514-t515+t523+t555-t583+t591+t603+t626+t670+t671+t680+t688+t25.*t157+t10.*t421+t25.*t465+t25.*t497+t10.*t23.*t421+t10.*t11.*t541+t5.*t10.*t25.*t58-t6.*t9.*t10.*t11.*t49.*2.0-t5.*t6.*t11.*t23.*t48.*2.0-dq1.*dq4.*t5.*t8.*t10.*t25.*2.0];
mt24 = [t51+t115+t120+t128+t207+t209+t220-t248+t294+t299-t333+t335+t340-t358+t375+t381-t383+t387+t389-t393-t414-t455+t476-t537+t540+t552-t554-t567-t589-t596+t604-t607-t612+t646-t651+t656+t672-t682+t683+t689-t25.*t207.*2.0+t6.*t11.*t24.*t58-t4.*t6.*t9.*t11.*t48.*4.0-t5.*t6.*t10.*t11.*t125.*2.0,t86+ddq3.*t3+ddq2.*t8.*4.318e-1+t3.*t13.*4.318e-1-dq2.*dq3.*t8.*2.0-ddq2.*q3.*t8-q3.*t3.*t13,t39.*t422.*(-2.0e-4),t32,0.0,0.0,0.0];
mt25 = [ddq1+t41+t50+t105+t107+t116+t127+t192+t193+t222+t223+t233+t288+t290+t311+t315+t324+t342+t343+t344+t418+t424+t431+t443+t472+t478+t480+t484+t493+t503+t509+t531+t542+t580+t585+t586+t647+t652+t653+t654-ddq6.*t8.*t10+ddq6.*t3.*t4.*t5,t47+t94+t118+t121+t126+t132+t205+t212+t227+t276+t328+t370+t394+t399+t420+t423+t427+t430+t466+t467+t483+t490+t507+t579+t584+t599+ddq6.*t5.*t9,0.0,ddq4+t39+t46+t48+t110+t114+t135+t194+t211+t219+t275+t308+t314+t327+t417+t447+t471+t496+t576+t601+t634-ddq6.*t10,t52+t103+t122+t129+t210+t216+t224+t258+t332+t345+t351+t373+t410+t428+t429+t465+t497+t515+t583+t602,ddq6+t70+t87+t115+t134+t136+t161+t220+t221+t226+t339+t340+t341,-t33+t54+t23.*t33.*2.0-t23.*t54.*2.0+t8.*t289+dq1.*dq4.*t22.*2.0-t3.*t4.*t45.*4.0-t4.*t9.*t91.*2.0-dq1.*dq4.*t22.*t23.*4.0];
mt26 = [-t32-dq2.*dq4.*2.0+t9.*t34.*2.0+t23.*t32.*2.0-t9.*t113.*4.0-t9.*t284.*2.0+dq2.*dq4.*t23.*4.0,0.0,t13+t273+t274+t289+t488,0.0,0.0,t60+t79-t102+t174-t177+t200+t242-t302,t42+t77+t98+t100+t185-t320,0.0,t40+t59+t297-dq1.*dq2.*t4.*t8.*2.0,0.0,0.0,-g.*t7,0.0,0.0,0.0,0.0,0.0,et39+et40,et68+et69,0.0];
mt27 = [t46+t53+t114+t117+t131-t211+t238+t240+t241-t250-t262-t300+t301+t331-t355-t359+t362+t367-t409+t437+t458-t475+t495+t498-t508+t524-t538+t556+t563+t590+t592-t597+t605+t650+t667+t678-t684-t10.*t25.*t51.*2.0+t6.*t11.*t85-t10.*t25.*t120.*2.0+t6.*t11.*t155-t10.*t25.*t207.*2.0+t24.*t25.*t495-t5.*t6.*t11.*t125.*2.0+t5.*t6.*t11.*t465-t4.*t6.*t9.*t11.*t119.*4.0-dq1.*dq6.*t6.*t8.*t11.*t24.*2.0-dq1.*dq5.*t3.*t6.*t9.*t10.*t11.*2.0];
mt28 = [ddq5+t34+t52-t97+t103+t111+t122+t125+t129-t148+t157-t164+t210+t216-t249-t253+t259-t267+t282+t295+t352-t361+t378-t380+t382-t397-t415-t456+t514+t533+t543-t555+t565+t606+t629+t637-t680-t24.*t25.*t45.*2.0-t24.*t25.*t113.*2.0-t24.*t25.*t125.*2.0+t10.*t25.*t421-t5.*t6.*t11.*t48.*2.0+t10.*t23.*t25.*t421+t4.*t9.*t11.*t492-t4.*t5.*t9.*t25.*t119.*2.0-dq2.*dq4.*t4.*t6.*t10.*t11.*2.0];
mt29 = [-t115+t119+t134+t208+t221+t226+t248-t294-t299+t333-t335+t339+t341+t358+t379-t381+t383-t387-t389+t393+t414+t440+t455+t517+t537+t547-t552+t554+t561+t567+t589+t596+t607+t612+t630+t651-t656-t672+t682-t25.*t561.*2.0+t6.*t11.*t273-t6.*t11.*t13.*t23.*2.0+t6.*t11.*t24.*t273+t6.*t11.*t23.*t24.*t273,t8.*t34-t3.*t42-t8.*t65.*2.0-t3.*t100-t8.*t113.*2.0+dq1.*dq2.*t9.*2.0+t3.*t4.*t13-dq1.*dq2.*t9.*t22.*4.0,ddq4.*t4-t9.*t14+t4.*t39+t9.*t58+t9.*t150.*2.0-dq1.*dq4.*t8.*t9.*2.0,0.0,t34+t125.*2.0+t157+t284,0.0,0.0,-g.*t3.*t7,-t76,0.0,0.0,0.0,0.0,t163,t64,0.0,0.0,0.0,0.0];
mt30 = [t50+t91+t127+t159+t203+t217+t270+t298+t323+t384+t388+t419,t36+t49+t93+t104+t204+t225+t269+t322+t329+t494,0.0,t46+t114+t131+t176+t240+t495,ddq5+t34+t103+t125+t157+t216,0.0,-ddq1.*t26-dq1.*dq2.*t21.*2.0,t12.*t21,0.0,0.0,0.0,0.0,t86,0.0,0.0,0.0,0.0,0.0,ddq1+t41+t50+t105+t107+t116+t127+t192+t193+t233+t288+t290+t311+t315+t324+t418+t424+t431+t443+t472+t478+t480+t484+t493+t503+t509+t531+t542+t580+t585+t586+t647+t652+t653+t654,t47+t94+t126+t132+t205+t276+t328+t370+t394+t399+t420+t423+t427+t430+t466+t467+t483+t490+t507+t579+t584+t599,0.0,ddq4+t39+t46+t48+t110+t114+t194+t275+t308+t314+t327+t417+t447+t471+t496+t576+t601+t634,t103+t216+t224+t258+t332+t345+t351+t373+t410+t428+t429+t465+t497+t515+t583+t602,0.0,t33-t54,t32,0.0,0.0,0.0,0.0,t133+t142+t232+t244+t469+t477+t479,t138+t187+t198+t369+ddq2.*t31+t31.*t132,0.0];
mt31 = [t48-t176+t321+t372,0.0,0.0,ddq2.*t8+t3.*t13,t39,0.0,0.0,0.0,0.0,t270+t298+t388+t31.*t50+t31.*t91+t23.*t133-t8.*t31.*t48.*2.0,t93-t187+t199+t269+t23.*t132+t3.*t8.*t12.*t31,0.0,t131+t176+t240+t495,0.0,0.0,t183+ddq1.*t30,t427,0.0,0.0,0.0,0.0,t91-t183,t329,0.0,0.0,0.0,0.0];
Yb = reshape([mt1,mt2,mt3,mt4,mt5,mt6,mt7,mt8,mt9,mt10,mt11,mt12,mt13,mt14,mt15,mt16,mt17,mt18,mt19,mt20,mt21,mt22,mt23,mt24,mt25,mt26,mt27,mt28,mt29,mt30,mt31],6,35);
end
